simulink library "thc"  (R2021b)
settings: Solver=VariableStepAuto  StartTime=0.0  StopTime=10.0  RelTol=1e-3
undefined symbols (not defined in the file or in its folder): ATHC_APTCQA_X_C, ATHC_APTCQB_X_C, ATHC_dAy_X_C, ATHC_Qeq_X_kmh, ATHC_VbaseC_X_C, ATHC_VbaseC_Y_W, ATHC_VbaseD_X_C, ATHC_VbaseH_X_C, KTHC_ACMaxMinT_sec, KTHC_aDeice_K, KTHC_AGSDefLv_K, KTHC_AGSLv1_K, KTHC_AGSLv2_K, KTHC_AGSLv3_K, KTHC_AGSLv4_K, KTHC_AGSLv5_K, KTHC_AirIntUpdateT_sec, KTHC_APTCOneZoneMax_W, KTHC_APTCPeriod_cnt, KTHC_APTCPWMEN_flg, KTHC_APTCQMaxC_W, KTHC_APTCQminC_W, KTHC_APTCQminD_W, KTHC_APTCQminRe1_W, KTHC_APTCQminRe_W, KTHC_APTCQoffT_cnt, KTHC_APTCQonT_cnt, KTHC_APTCRiLeMaxDff_W, KTHC_APTCRiLeMinDff_W, KTHC_AutoWDTamb1_C, KTHC_AutoWDTamb2_C, KTHC_AutoWDTamb3_C, KTHC_BatCoolT_cnt, KTHC_BatInTempDef_C, KTHC_bDeice_K, KTHC_CompMaxDeice_rpm, KTHC_CompMinDeice_rpm, KTHC_CompSotxvOp_K, KTHC_CompSotxvOpLow_rpm, KTHC_CompSpdEXVUp1_rpm, KTHC_CompSpdEXVUp2_rpm, KTHC_CompSpdEXVUp3_rpm, KTHC_CompSpdEXVUp4_rpm, KTHC_CompSpdmax_rpm, KTHC_CompSpdmaxBC1_rpm, KTHC_CompSpdmaxBC_rpm, KTHC_CompSpdmid1_rpm, KTHC_CompSpdmid2_rpm, KTHC_CompSpdmid3_rpm, KTHC_CompSpdmid4_rpm, KTHC_CompSpdmid5_rpm, KTHC_CompSpdmid_rpm, KTHC_CompSpdmin_rpm, KTHC_DAPTCQ1_W, KTHC_DAPTCQ2_W, KTHC_DAPTCQ3_W, KTHC_DcChSetTemp_C, KTHC_DehumidityEN_flg, KTHC_DeiceCycTime_K, KTHC_DriveLevelWPTCBAH1_W ... (+403)
libraries: simulink x489
(part 3 of 18)

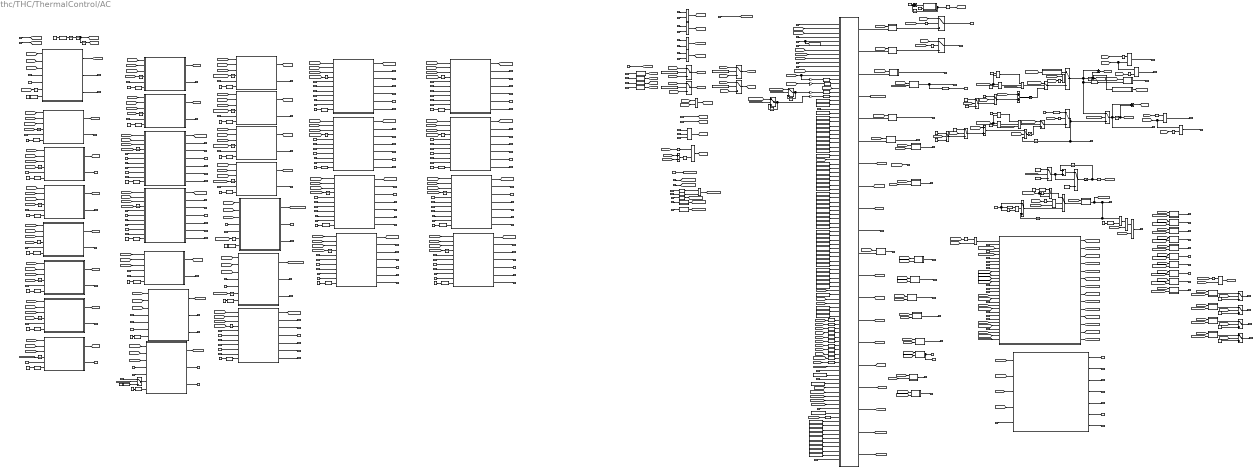
== system thc/THC/ThermalControl/AC ==
  note: PersonalSetting
  VINP_FCPFrEvtBtnACMaxReq_flg : Inport
  VINP_FCPFrEvtBtnACReq_flg : Inport  Port=2
  VINP_FCPFrEvtBtnAutoReq_flg : Inport  Port=3
  VINP_FCPFrEvtBtnSyncReq_flg : Inport  Port=4
  VINP_Tamb_C : Inport  Port=5
  VINP_Tincar_C : Inport  Port=6
  VINP_sigAirIntenZon1Req_enum : Inport  Port=7
  VINP_sigRecircReq_flg : Inport  Port=8
  VINP_sigFaceReq_flg : Inport  Port=9
  VINP_sigFootReq_flg : Inport  Port=10
  VINP_sigFrostReq_flg : Inport  Port=11
  VINP_sigSetTempZon1Req_C : Inport  Port=12
  VINP_CANMsgValidIVI2_flg : Inport  Port=13
  VINP_sigSetTempZon2Req_C : Inport  Port=14
  VTHC_FDBlowerCmd_pct : Inport  Port=15
  PwrSta : Inport  Port=16
  OFF_AC_MODE : Inport  Port=17
  CabinMode : Inport  Port=18
  T_Foot_L : Inport  Port=19
  T_Foot_R : Inport  Port=20
  T_Foot_Rr : Inport  Port=21
  VINP_RemoteAutoReq_flg : Inport  Port=22
  ACSubMode : Inport  Port=23
  EEP_sigSetTempZon2StM : Inport  Port=24
  VINP_HMIACBtnCmd_flg : Inport  Port=25
  VINP_HMIACAutoBtnCmd_flg : Inport  Port=26
  VINP_HMIACRecycleBtnCmd_flg : Inport  Port=27
  VINP_HMIACFrDefogBtnCmd_flg : Inport  Port=28
  VINP_HMIZLSetTPCmd_flg : Inport  Port=29
  VINP_HMIZLSetTMCmd_flg : Inport  Port=30
  VINP_HMIZRSetTPCmd_flg : Inport  Port=31
  VINP_HMIZRSetTMCmd_flg : Inport  Port=32
  VINP_HMIACWindDirPCmd_flg : Inport  Port=33
  VINP_HMIACWindDirMCmd_flg : Inport  Port=34
  VINP_HMIACAirIntPCmd_flg : Inport  Port=35
  VINP_HMIACAirIntMCmd_flg : Inport  Port=36
  VINP_IVIAirIntZ3Cmd_enum : Inport  Port=37
  VINP_IVILBlowerModeSta_enum : Inport  Port=38
  VINP_IVIRBlowerModeSta_enum : Inport  Port=39
  VINP_IVILBlowerZSta_enum : Inport  Port=40
  VINP_IVICLBlowerZSta_enum : Inport  Port=41
  VINP_IVIRBlowerZSta_enum : Inport  Port=42
  VINP_IVICRBlowerZSta_enum : Inport  Port=43
  VINP_IVILBlowerYSta_enum : Inport  Port=44
  VINP_IVICLBlowerYSta_enum : Inport  Port=45
  VINP_IVIRBlowerYSta_enum : Inport  Port=46
  VINP_IVICRBlowerYSta_enum : Inport  Port=47
  VINP_ZFRTHCLEventActYSta_enum : Inport  Port=48
  VINP_ZFRTHCCLEVentActYSta_enum : Inport  Port=49
  VINP_ZFRTHCREventActYSta_enum : Inport  Port=50
  VINP_ZFRTHCCREVentActYSta_enum : Inport  Port=51
  VINP_IVIsigScreenReq_Sta : Inport  Port=52
  VINP_IVIFGSAirIntCmd_enum : Inport  Port=53
  VINP_IVIFGSChCmd_enum : Inport  Port=54
  VINP_IVIIONSWCmd_flg : Inport  Port=55
  VINP_FGSAirIntSta_enum : Inport  Port=56
  VINP_IVIZon1WindDirSWReqSta_flg : Inport  Port=57
  VBCM_UserNow_enum : Inport  Port=58
  VINP_UpdateReq_enum : Inport  Port=59
  EEP_ACModeSet123 : Inport  Port=60
  EEP_ACModeSet457 : Inport  Port=61
  EEP_FACESet : Inport  Port=62
  EEP_FOOTSet : Inport  Port=63
  EEP_FrostSet : Inport  Port=64
  EEP_FaceMSet : Inport  Port=65
  EEP_FootMSet : Inport  Port=66
  EEP_fdefogSet : Inport  Port=67
  EEP_CCUSyncStsSet : Inport  Port=68
  EEP_sigRecircStSet : Inport  Port=69
  EEP_RecyAutoSet : Inport  Port=70
  EEP_AirIntenZone1MSet1 : Inport  Port=71
  EEP_AirIntenZone1MSet2 : Inport  Port=72
  EEP_AirIntenZone1MSet3 : Inport  Port=73
  EEP_AirIntenZone1MSet4 : Inport  Port=74
  EEP_AirIntenZone1MSet5 : Inport  Port=75
  EEP_AirIntenZone1MSet7 : Inport  Port=76
  EEP_AirIntenZone3MSet1 : Inport  Port=77
  EEP_AirIntenZone3MSet2 : Inport  Port=78
  EEP_AirIntenZone3MSet3 : Inport  Port=79
  EEP_AirIntenZone3MSet4 : Inport  Port=80
  EEP_AirIntenZone3MSet5 : Inport  Port=81
  EEP_AirIntenZone3MSet7 : Inport  Port=82
  EEP_IONSWStaSet : Inport  Port=83
  EEP_FDCFGSChStaSet123 : Inport  Port=84
  EEP_FDCFGSChStaSet457 : Inport  Port=85
  EEP_FDCFGSAirIntStaSet123 : Inport  Port=86
  EEP_FDCFGSAirIntStaSet457 : Inport  Port=87
  EEP_LVentENSet : Inport  Port=88
  EEP_CLVentENSet : Inport  Port=89
  EEP_RVentENSet : Inport  Port=90
  EEP_CRVentENSet : Inport  Port=91
  EEP_FDCTHCLEventModeStaSet123 : Inport  Port=92
  EEP_FDCTHCLEventModeStaSet457 : Inport  Port=93
  EEP_FDCTHCREventModeStaSet123 : Inport  Port=94
  EEP_FDCTHCREventModeStaSet457 : Inport  Port=95
  EEP_FDCTHCLEventZStaSet1 : Inport  Port=96
  EEP_FDCTHCLEventZStaSet2 : Inport  Port=97
  EEP_FDCTHCLEventZStaSet3 : Inport  Port=98
  EEP_FDCTHCLEventZStaSet4 : Inport  Port=99
  EEP_FDCTHCLEventZStaSet5 : Inport  Port=100
  EEP_FDCTHCLEventZStaSet7 : Inport  Port=101
  EEP_FDCTHCCLEVentZStaSet1 : Inport  Port=102
  EEP_FDCTHCCLEVentZStaSet2 : Inport  Port=103
  EEP_FDCTHCCLEVentZStaSet3 : Inport  Port=104
  EEP_FDCTHCCLEVentZStaSet4 : Inport  Port=105
  EEP_FDCTHCCLEVentZStaSet5 : Inport  Port=106
  EEP_FDCTHCCLEVentZStaSet7 : Inport  Port=107
  EEP_FDCTHCREventZStaSet1 : Inport  Port=108
  EEP_FDCTHCREventZStaSet2 : Inport  Port=109
  EEP_FDCTHCREventZStaSet3 : Inport  Port=110
  EEP_FDCTHCREventZStaSet4 : Inport  Port=111
  EEP_FDCTHCREventZStaSet5 : Inport  Port=112
  EEP_FDCTHCREventZStaSet7 : Inport  Port=113
  EEP_FDCTHCCREVentZStaSet1 : Inport  Port=114
  EEP_FDCTHCCREVentZStaSet2 : Inport  Port=115
  EEP_FDCTHCCREVentZStaSet3 : Inport  Port=116
  EEP_FDCTHCCREVentZStaSet4 : Inport  Port=117
  EEP_FDCTHCCREVentZStaSet5 : Inport  Port=118
  EEP_FDCTHCCREVentZStaSet7 : Inport  Port=119
  EEP_FDCTHCLEventYStaSet1 : Inport  Port=120
  EEP_FDCTHCLEventYStaSet2 : Inport  Port=121
  EEP_FDCTHCLEventYStaSet3 : Inport  Port=122
  EEP_FDCTHCLEventYStaSet4 : Inport  Port=123
  EEP_FDCTHCLEventYStaSet5 : Inport  Port=124
  EEP_FDCTHCLEventYStaSet7 : Inport  Port=125
  EEP_FDCTHCCLEVentYStaSet1 : Inport  Port=126
  EEP_FDCTHCCLEVentYStaSet2 : Inport  Port=127
  EEP_FDCTHCCLEVentYStaSet3 : Inport  Port=128
  EEP_FDCTHCCLEVentYStaSet4 : Inport  Port=129
  EEP_FDCTHCCLEVentYStaSet5 : Inport  Port=130
  EEP_FDCTHCCLEVentYStaSet7 : Inport  Port=131
  EEP_FDCTHCREventYStaSet1 : Inport  Port=132
  EEP_FDCTHCREventYStaSet2 : Inport  Port=133
  EEP_FDCTHCREventYStaSet3 : Inport  Port=134
  EEP_FDCTHCREventYStaSet4 : Inport  Port=135
  EEP_FDCTHCREventYStaSet5 : Inport  Port=136
  EEP_FDCTHCREventYStaSet7 : Inport  Port=137
  EEP_FDCTHCCREVentYStaSet1 : Inport  Port=138
  EEP_FDCTHCCREVentYStaSet2 : Inport  Port=139
  EEP_FDCTHCCREVentYStaSet3 : Inport  Port=140
  EEP_FDCTHCCREVentYStaSet4 : Inport  Port=141
  EEP_FDCTHCCREVentYStaSet5 : Inport  Port=142
  EEP_FDCTHCCREVentYStaSet7 : Inport  Port=143
  EEP_SettempZon1Set1 : Inport  Port=144
  EEP_SettempZon1Set2 : Inport  Port=145
  EEP_SettempZon1Set3 : Inport  Port=146
  EEP_SettempZon1Set4 : Inport  Port=147
  EEP_SettempZon1Set5 : Inport  Port=148
  EEP_SettempZon1Set7 : Inport  Port=149
  VINP_IVIQuickRefreshSta_flg : Inport  Port=150
  Add{,1..2,5} (4 alike) : Sum
  Add3 : Sum  Inputs=+-
  Add7 : Sum  Inputs=+-
  Add8 : Sum  Inputs=+-
  Chart : Stateflow chart  TreatAsAtomicUnit=on
      settings: PortSchema="{\"entries\":[{\"content\":{\"sides\":[{\"content\":{\"connectorIds\":[\"In1\",\"In2\",\"In3\",\"In4\",\"In5\",\"In6\",\"In7\",\"In8\",\"In9\",\"In10\",\"In11\",\"In12\",\"In13\",\"In14\",\"In15\",\"In16\",\"In18\",\"In17\",\"In19\",\"In20\",\"In21\",\"In22\",\"In23\",\"In24\",\"In25\",\"In26\",\"In27\",\"In28\",\"In29\",\"In30\",\"In31\",\"In32\",\"In33\",\"In34\",\"In35\",\"In36\",\"In37\",\"In38\",\"In39\",\"In40\",\"In41\",\"In42\",\"In43\",\"In44\",\"In45\",\"In46\",\"In47\",\"In48\",\"In49\",\"In50\",\"In51\",\"In52\",\"In53\",\"In54\",\"In55\",\"In56\",\"In57\",\"In58\",\"In59\",\"In60\",\"In61\",\"In62\",\"In63\",\"In64\",\"In65\",\"In66\",\"In67\",\"In68\",\"In69\",\"In70\",\"In71\",\"In72\",\"In73\",\"In74\",\"In75\",\"In76\",\"In77\",\"In78\",\"In79\",\"In80\",\"In81\",\"In82\",\"In83\",\"In84\",\"In85\",\"In86\",\"In87\",\"In88\",\"In89\",\"In90\",\"In91\",\"In92\",\"In93\",\"In94\",\"In95\",\"In96\",\"In97\",\"In98\",\"In99\",\"In100\",\"In101\",\"In102\",\"In103\",\"In104\"]},\"type\":\"ConnectorPlacement.EquallySpacedRectSide\",\"uuid\":\"5820fc40-35f0-4b43-a348-a95be02a5108\"},{\"content\":{\"connectorIds\":[\"Out1\",\"Out6\",\"Out2\",\"Out3\",\"Out4\",\"Out5\",\"Out7\",\"Out8\",\"Out9\",\"Out10\",\"Out11\",\"Out12\",\"Out13\",\"Out14\",\"Out15\",\"Out16\",\"Out17\",\"Out18\",\"Out19\",\"Out20\"],\"side\":\"RIGHT\"},\"type\":\"ConnectorPlacement.EquallySpacedRectSide\",\"uuid\":\"36d6613c-bf09-4a00-b7cd-6c94d14300cf\"},{\"content\":{\"connectorIds\":[],\"side\":\"TOP\"},\"type\":\"ConnectorPlacement.EquallySpacedRectSide\",\"uuid\":\"1ae2c247-46e8-45cc-9ea1-ac445f4d9fda\"}]},\"type\":\"ConnectorPlacement.EquallySpacedConnector\",\"uuid\":\"a8684177-dc23-416a-a392-32f98192c4b4\"}],\"packageUris\":[\"http://schema.mathworks.com/mf0/Connector/R2020b\"],\"version\":\"1.0\"}"
  Compare To Constant : simulink/Logic and Bit Operations/Compare To Constant  relop=<  const=5  OutDataTypeStr=boolean
  Compare To Constant1 : simulink/Logic and Bit Operations/Compare To Constant  relop=>=  const=1  OutDataTypeStr=boolean
  Compare To Constant10 : simulink/Logic and Bit Operations/Compare To Constant  relop=>  const=0  OutDataTypeStr=boolean
  Compare To Constant11 : simulink/Logic and Bit Operations/Compare To Constant  relop=<  const=0  OutDataTypeStr=boolean
  Compare To Constant12 : simulink/Logic and Bit Operations/Compare To Constant  relop=>  const=0  OutDataTypeStr=boolean
  Compare To Constant13 : simulink/Logic and Bit Operations/Compare To Constant  relop=<  const=0  OutDataTypeStr=boolean
  Compare To Constant2 : simulink/Logic and Bit Operations/Compare To Constant  relop=>=  const=100  OutDataTypeStr=boolean
  Compare To Constant3 : simulink/Logic and Bit Operations/Compare To Constant  relop===  const=3.0  OutDataTypeStr=boolean
  Compare To Constant4 : simulink/Logic and Bit Operations/Compare To Constant  relop=<  const=0  OutDataTypeStr=boolean
  Compare To Constant6 : simulink/Logic and Bit Operations/Compare To Constant  relop===  const=2  OutDataTypeStr=boolean
  Compare To Constant7 : simulink/Logic and Bit Operations/Compare To Constant  relop===  const=1  OutDataTypeStr=boolean
  Compare To Constant8 : simulink/Logic and Bit Operations/Compare To Constant  relop===  const=0  OutDataTypeStr=boolean
  Compare To Constant9 : simulink/Logic and Bit Operations/Compare To Constant  relop=>  const=0  OutDataTypeStr=boolean
  Constant{,55,71,80,82,85,91,94,96..101} (14 alike) : Constant
  Constant1 : Constant  Value=10
  Constant10 : Constant  Value=KTHC_T2Mmaxamb_C
  Constant{102..109} (8 alike) : Constant  Value=50
  Constant11 : Constant  Value=KTHC_T3Mmaxamb_C
  Constant{68..70,110} (4 alike) : Constant  Value=KTHC_DriverSeatPos_flg
  Constant111 : Constant  Value=KTHC_AutoWDTamb1_C
  Constant112 : Constant  Value=KTHC_AutoWDTamb2_C
  Constant113 : Constant  Value=KTHC_AutoWDTamb3_C
  Constant114 : Constant  Value=KTHC_WDZ11Foot_flg
  Constant115 : Constant  Value=KTHC_WDZ11Frost_flg
  Constant116 : Constant  Value=KTHC_WDZ11Face_flg
  Constant117 : Constant  Value=KTHC_WDZ12Foot_flg
  Constant118 : Constant  Value=KTHC_WDZ12Frost_flg
  Constant119 : Constant  Value=KTHC_WDZ12Face_flg
  Constant12 : Constant  Value=KTHC_T4Mmaxamb_C
  Constant13 : Constant  Value=KTHC_T3Mminamb_C
  Constant14 : Constant  Value=KTHC_T4Mminamb_C
  Constant15 : Constant  Value=KTHC_T5Mminamb_C
  Constant16 : Constant  Value=KTHC_RecyHold_min
  Constant17 : Constant  Value=KTHC_RecyChange_min
  Constant18 : Constant  Value=KTHC_Tmidlevel_C
  Constant19 : Constant  Value=KTHC_Thilevel1_C
  Constant20 : Constant  Value=KTHC_Thilevel2_C
  Constant21 : Constant  Value=KTHC_WDZ1Face_flg
  Constant22 : Constant  Value=KTHC_WDZ1Foot_flg
  Constant23 : Constant  Value=KTHC_WDZ1Frost_flg
  Constant24 : Constant  Value=KTHC_WDZ2Face_flg
  Constant25 : Constant  Value=KTHC_WDZ2Foot_flg
  Constant26 : Constant  Value=KTHC_WDZ2Frost_flg
  Constant27 : Constant  Value=KTHC_WDZ3Face_flg
  Constant28 : Constant  Value=KTHC_WDZ3Foot_flg
  Constant29 : Constant  Value=KTHC_WDZ3Frost_flg
  Constant30 : Constant  Value=KTHC_WDZ4Face_flg
  Constant31 : Constant  Value=KTHC_WDZ4Foot_flg
  Constant32 : Constant  Value=KTHC_WDZ4Frost_flg
  Constant33 : Constant  Value=KTHC_WDZ5Face_flg
  Constant34 : Constant  Value=KTHC_WDZ5Foot_flg
  Constant35 : Constant  Value=KTHC_WDZ5Frost_flg
  Constant36 : Constant  Value=KTHC_WDZ6Face_flg
  Constant37 : Constant  Value=KTHC_WDZ6Foot_flg
  Constant38 : Constant  Value=KTHC_WDZ6Frost_flg
  Constant39 : Constant  Value=KTHC_WDZ7Face_flg
  Constant4 : Constant  Value=ZERO_INT
  Constant40 : Constant  Value=KTHC_WDZ7Foot_flg
  Constant41 : Constant  Value=KTHC_WDZ7Frost_flg
  Constant42 : Constant  Value=KTHC_WDZ8Face_flg
  Constant43 : Constant  Value=KTHC_WDZ8Foot_flg
  Constant44 : Constant  Value=KTHC_WDZ8Frost_flg
  Constant45 : Constant  Value=KTHC_WDZ9Face_flg
  Constant46 : Constant  Value=KTHC_WDZ9Foot_flg
  Constant47 : Constant  Value=KTHC_WDZ9Frost_flg
  Constant48 : Constant  Value=ONE_INT
  Constant49 : Constant  Value=ZERO_INT
  Constant5 : Constant  Value=KTHC_RecyOutterD_enum
  Constant50 : Constant  Value=KTHC_Trecymin_C
  Constant51 : Constant  Value=KTHC_RefreshEN_flg
  Constant52 : Constant  Value=KTHC_FootColdT_C
  Constant53 : Constant  Value=KTHC_FootColdTdelta_C
  Constant54 : Constant  Value=KTHC_ACMaxMinT_sec
  Constant57 : Constant  Value=KTHC_WDZ10Foot_flg
  Constant58 : Constant  Value=KTHC_WDZ10Frost_flg
  Constant59 : Constant  Value=0.5
  Constant6 : Constant  Value=KTHC_WDZ10Face_flg
  Constant60 : Constant  Value=-0.5
  Constant{61,64,81,83..84,86..90,93,95} (12 alike) : Constant  Value=0
  Constant62 : Constant  Value=0.5
  Constant63 : Constant  Value=-0.5
  Constant65 : Constant  Value=32
  Constant66 : Constant  Value=32
  Constant67 : Constant  Value=7
  Constant7 : Constant  Value=KTHC_WindDirUpdateT_min
  Constant{72..75} (4 alike) : Constant  Value=false
  Constant76 : Constant  Value=4
  Constant77 : Constant  Value=17
  Constant78 : Constant  Value=17
  Constant79 : Constant  Value=KTHC_ScreenUniq_flg
  Constant9 : Constant  Value=KTHC_AirIntUpdateT_sec
  Constant92 : Constant  Value=4
  Data Type Conversion : DataTypeConversion
  Data Type Conversion1 : DataTypeConversion  OutDataTypeStr=single
  Data Type Conversion{6..7,10..11,24..25,27..28,33..43,50} (20 alike) : DataTypeConversion  OutDataTypeStr=uint8
  Data Type Conversion12 : DataTypeConversion  OutDataTypeStr=single
  Data Type Conversion{8..9,13,15..23,26,29..32,44..49,51} (24 alike) : DataTypeConversion  OutDataTypeStr=boolean
  Data Type Conversion{2..5,14} (5 alike) : DataTypeConversion  OutDataTypeStr=uint16
  Detect Change : simulink/Logic and Bit Operations/Detect Change  vinit=0  OutDataTypeStr=boolean
  Detect Change1 : simulink/Logic and Bit Operations/Detect Change  vinit=0  OutDataTypeStr=boolean
  Detect Increase4 : simulink/Logic and Bit Operations/Detect Increase  vinit=0.0  OutDataTypeStr=boolean
  Detect Increase5 : simulink/Logic and Bit Operations/Detect Increase  vinit=0.0  OutDataTypeStr=boolean
  Detect Increase7 : simulink/Logic and Bit Operations/Detect Increase  vinit=0.0  OutDataTypeStr=boolean
  EVent : Subsystem
  Gain{,1..3} (4 alike) : Gain  Gain=10
  HMISwitchReceive : Subsystem
  HMISwitchReceive1 : Subsystem
  HMISwitchReceive2 : Subsystem
  HMISwitchReceive3 : Subsystem
  HMISwitchReceive4 : Subsystem
  HMISwitchReceive5 : Subsystem
  Logical Operator : Logic  Operator=NXOR  AllPortsSameDT=off  OutDataTypeStr=boolean
  Logical Operator{1..2,4..6,11,20..21,23} (9 alike) : Logic  Operator=OR  AllPortsSameDT=off  OutDataTypeStr=boolean
  Logical Operator{3,10,12..16,22} (8 alike) : Logic  AllPortsSameDT=off  OutDataTypeStr=boolean
  Logical Operator{9,25..27} (4 alike) : Logic  Operator=NOT  AllPortsSameDT=off  OutDataTypeStr=boolean
  Logical Operator7 : Logic  Inputs=3  AllPortsSameDT=off  OutDataTypeStr=boolean
  Logical Operator8 : Logic  Inputs=3  AllPortsSameDT=off  OutDataTypeStr=boolean
  Min : MinMax  Inputs=3
  ModMath2 : Subsystem  mask(Count){}
      mask help: Counter function.
      mask Display:
      | fprintf('ModMath');
      | port_label('output', 1, 'Remainder');
      | port_label('input', 1, 'Dividend');
      | port_label('input', 2, 'Divisor');
  RawdataToSettemp : Subsystem
  Relational Operator{,1,4..5} (4 alike) : RelationalOperator  Operator=<=  OutDataTypeStr=boolean  RndMeth=Simplest
  Relational Operator3 : RelationalOperator  Operator=>  OutDataTypeStr=boolean  RndMeth=Simplest
  Saturation : Saturate  UpperLimit=100  LowerLimit=0
  Saturation2 : Saturate  UpperLimit=32  LowerLimit=17
  Saturation3 : Saturate  UpperLimit=32  LowerLimit=17
  SettempToRawData : Subsystem
  Subsystem : Subsystem
  Subsystem1 : Subsystem
  Subsystem10 : Subsystem
  Subsystem11 : Subsystem
  Subsystem12 : Subsystem
  Subsystem13 : Subsystem
  Subsystem14 : Subsystem
  Subsystem15 : Subsystem
  Subsystem16 : Subsystem
  Subsystem17 : Subsystem
  Subsystem18 : Subsystem
  Subsystem19 : Subsystem
  Subsystem2 : Subsystem
  Subsystem20 : Subsystem
  Subsystem21 : Subsystem
  Subsystem22 : Subsystem
  Subsystem23 : Subsystem
  Subsystem24 : Subsystem
  Subsystem25 : Subsystem
  Subsystem26 : Subsystem
  Subsystem27 : Subsystem
  Subsystem28 : Subsystem
  Subsystem29 : Subsystem
  Subsystem3 : Subsystem
  Subsystem30 : Subsystem
  Subsystem31 : Subsystem
  Subsystem32 : Subsystem
  Subsystem33 : Subsystem
  Subsystem4 : Subsystem
  Subsystem5 : Subsystem
  Subsystem6 : Subsystem
  Subsystem7 : Subsystem
  Subsystem8 : Subsystem
  Subsystem9 : Subsystem
  Switch{,1..3,9..32} (28 alike) : Switch  Criteria=u2 > Threshold
  TOGGLE_TYPE_CCUSyncSts : Subsystem
  TOGGLE_TYPE_CLVentEN : Subsystem
  TOGGLE_TYPE_CRVentEN : Subsystem
  TOGGLE_TYPE_FACE : Subsystem
  TOGGLE_TYPE_FACEM : Subsystem
  TOGGLE_TYPE_FOOT : Subsystem
  TOGGLE_TYPE_FOOTM : Subsystem
  TOGGLE_TYPE_FROST : Subsystem
  TOGGLE_TYPE_IONSWSta : Subsystem
  TOGGLE_TYPE_LVentEN : Subsystem
  TOGGLE_TYPE_RVentEN : Subsystem
  TOGGLE_TYPE_RecyAutoFlg : Subsystem
  TOGGLE_TYPE_fdefog : Subsystem
  TOGGLE_TYPE_sigRecircSt : Subsystem
  Unit Delay1 : UnitDelay  InitialCondition=26  SampleTime=-1  HasFrameUpgradeWarning=on
  Unit Delay{2..38} (37 alike) : UnitDelay  SampleTime=-1  HasFrameUpgradeWarning=on
  VALUE_TYPE_ACModeMem : Subsystem
  VALUE_TYPE_AirIntenZone1M : Subsystem
  VALUE_TYPE_AirIntenZone3M : Subsystem
  VALUE_TYPE_FDCFGSAirIntSta : Subsystem
  VALUE_TYPE_FDCFGSChStaSet : Subsystem
  VALUE_TYPE_FDCTHCCLEVentYSta : Subsystem
  VALUE_TYPE_FDCTHCCLEVentZSta : Subsystem
  VALUE_TYPE_FDCTHCCREVentYSta : Subsystem
  VALUE_TYPE_FDCTHCCREVentZSta : Subsystem
  VALUE_TYPE_FDCTHCLEventYSta : Subsystem
  VALUE_TYPE_FDCTHCLEventZSta : Subsystem
  VALUE_TYPE_FDCTHCREventYSta : Subsystem
  VALUE_TYPE_FDCTHCREventZSta : Subsystem
  VALUE_TYPE_LEventModeSta : Subsystem
  VALUE_TYPE_REventModeSta : Subsystem
  VALUE_TYPE_SettempZon1 : Subsystem
  VTHC_CCUACLampSts_flg : Outport
  VTHC_CCUAutoLampSts_flg : Outport  Port=2
  VTHC_CCUACMaxLampSts_flg : Outport  Port=3
  VTHC_CCUSyncLampSts_flg : Outport  Port=4
  VTHC_sigAirIntenZon1St_enum : Outport  Port=5
  VTHC_sigWindDirZon1St_enum : Outport  Port=6
  VTHC_sigRecircSt_flg : Outport  Port=7
  VTHC_sigSetTempZon1St_C : Outport  Port=8
  VTHC_sigSetTempZon2St_C : Outport  Port=9
  WaterFillReq : Outport  Port=10
  PET : Outport  Port=11
  FD_RecyAuto_Cmd : Outport  Port=12
  ACModeMem : Outport  Port=13
  Face : Outport  Port=14
  Foot : Outport  Port=15
  Frost : Outport  Port=16
  FaceM : Outport  Port=17
  FootM : Outport  Port=18
  CCUSyncSts : Outport  Port=19
  RecAutoFlg : Outport  Port=20
  AirIntenZone1M : Outport  Port=21
  fdefog : Outport  Port=22
  VTHC_sigSetTempZon2StM_C : Outport  Port=23
  VTHC_sigDfrstSt_flg : Outport  Port=24
  VTHC_FDCTHCAirIntZ3Sta_enum : Outport  Port=25
  RrAPTCEN : Outport  Port=26
  VTHC_FDCTHCLEventModeSta_enum : Outport  Port=27
  VTHC_FDCTHCREventModeSta_enum : Outport  Port=28
  VTHC_FDCTHCLEventZSta_enum : Outport  Port=29
  VTHC_FDCTHCCLEVentZSta_enum : Outport  Port=30
  VTHC_FDCTHCREventZSta_enum : Outport  Port=31
  VTHC_FDCTHCCREVentZSta_enum : Outport  Port=32
  VTHC_FDCTHCLEventYSta_enum : Outport  Port=33
  VTHC_FDCTHCLVentENSta_flg : Outport  Port=34
  VTHC_FDCTHCCLEVentYSta_enum : Outport  Port=35
  VTHC_FDCTHCCLVentENSta_flg : Outport  Port=36
  VTHC_FDCTHCREventYSta_enum : Outport  Port=37
  VTHC_FDCTHCRVentENSta_flg : Outport  Port=38
  VTHC_FDCTHCCREVentYSta_enum : Outport  Port=39
  VTHC_FDCTHCCRVentENSta_flg : Outport  Port=40
  VTHC_Z1TUP_flg : Outport  Port=41
  VTHC_Z1TDN_flg : Outport  Port=42
  VTHC_Z2TUP_flg : Outport  Port=43
  VTHC_Z2TDN_flg : Outport  Port=44
  VTHC_FDCFGSAirIntSta_enum : Outport  Port=45
  VTHC_FDCFGSChSta_enum : Outport  Port=46
  VTHC_FDCFGSAirIntCmd_enum : Outport  Port=47
  VTHC_FDCFGSFuncSta_enum : Outport  Port=48
  VTHC_FDCFGSChCmd_enum : Outport  Port=49
  VTHC_FDCFGSIONSWSta_flg : Outport  Port=50
  VTHC_FDCFGSIONCmd_flg : Outport  Port=51
  ACModeSet123 : Outport  Port=52
  ACModeSet457 : Outport  Port=53
  FACESet : Outport  Port=54
  FOOTSet : Outport  Port=55
  FrostSet : Outport  Port=56
  FaceMSet : Outport  Port=57
  FootMSet : Outport  Port=58
  fdefogSet : Outport  Port=59
  CCUSyncStsSet : Outport  Port=60
  sigRecircStSet : Outport  Port=61
  RecyAutoSet : Outport  Port=62
  AirIntenZone1MSet1 : Outport  Port=63
  AirIntenZone1MSet2 : Outport  Port=64
  AirIntenZone1MSet3 : Outport  Port=65
  AirIntenZone1MSet4 : Outport  Port=66
  AirIntenZone1MSet5 : Outport  Port=67
  AirIntenZone1MSet7 : Outport  Port=68
  AirIntenZone3MSet1 : Outport  Port=69
  AirIntenZone3MSet2 : Outport  Port=70
  AirIntenZone3MSet3 : Outport  Port=71
  AirIntenZone3MSet4 : Outport  Port=72
  AirIntenZone3MSet5 : Outport  Port=73
  AirIntenZone3MSet7 : Outport  Port=74
  IONSWStaSet : Outport  Port=75
  FDCFGSChStaSet123 : Outport  Port=76
  FDCFGSChStaSet457 : Outport  Port=77
  FDCFGSAirIntStaSet123 : Outport  Port=78
  FDCFGSAirIntStaSet457 : Outport  Port=79
  LVentENSet : Outport  Port=80
  CLVentENSet : Outport  Port=81
  RVentENSet : Outport  Port=82
  CRVentENSet : Outport  Port=83
  FDCTHCLEventModeStaSet123 : Outport  Port=84
  FDCTHCLEventModeStaSet457 : Outport  Port=85
  FDCTHCREventModeStaSet123 : Outport  Port=86
  FDCTHCREventModeStaSet457 : Outport  Port=87
  FDCTHCLEventZStaSet1 : Outport  Port=88
  FDCTHCLEventZStaSet2 : Outport  Port=89
  FDCTHCLEventZStaSet3 : Outport  Port=90
  FDCTHCLEventZStaSet4 : Outport  Port=91
  FDCTHCLEventZStaSet5 : Outport  Port=92
  FDCTHCLEventZStaSet7 : Outport  Port=93
  FDCTHCCLEVentZStaSet1 : Outport  Port=94
  FDCTHCCLEVentZStaSet2 : Outport  Port=95
  FDCTHCCLEVentZStaSet3 : Outport  Port=96
  FDCTHCCLEVentZStaSet4 : Outport  Port=97
  FDCTHCCLEVentZStaSet5 : Outport  Port=98
  FDCTHCCLEVentZStaSet7 : Outport  Port=99
  FDCTHCREventZStaSet1 : Outport  Port=100
  FDCTHCREventZStaSet2 : Outport  Port=101
  FDCTHCREventZStaSet3 : Outport  Port=102
  FDCTHCREventZStaSet4 : Outport  Port=103
  FDCTHCREventZStaSet5 : Outport  Port=104
  FDCTHCREventZStaSet7 : Outport  Port=105
  FDCTHCCREVentZStaSet1 : Outport  Port=106
  FDCTHCCREVentZStaSet2 : Outport  Port=107
  FDCTHCCREVentZStaSet3 : Outport  Port=108
  FDCTHCCREVentZStaSet4 : Outport  Port=109
  FDCTHCCREVentZStaSet5 : Outport  Port=110
  FDCTHCCREVentZStaSet7 : Outport  Port=111
  FDCTHCLEventYStaSet1 : Outport  Port=112
  FDCTHCLEventYStaSet2 : Outport  Port=113
  FDCTHCLEventYStaSet3 : Outport  Port=114
  FDCTHCLEventYStaSet4 : Outport  Port=115
  FDCTHCLEventYStaSet5 : Outport  Port=116
  FDCTHCLEventYStaSet7 : Outport  Port=117
  FDCTHCCLEVentYStaSet1 : Outport  Port=118
  FDCTHCCLEVentYStaSet2 : Outport  Port=119
  FDCTHCCLEVentYStaSet3 : Outport  Port=120
  FDCTHCCLEVentYStaSet4 : Outport  Port=121
  FDCTHCCLEVentYStaSet5 : Outport  Port=122
  FDCTHCCLEVentYStaSet7 : Outport  Port=123
  FDCTHCREventYStaSet1 : Outport  Port=124
  FDCTHCREventYStaSet2 : Outport  Port=125
  FDCTHCREventYStaSet3 : Outport  Port=126
  FDCTHCREventYStaSet4 : Outport  Port=127
  FDCTHCREventYStaSet5 : Outport  Port=128
  FDCTHCREventYStaSet7 : Outport  Port=129
  FDCTHCCREVentYStaSet1 : Outport  Port=130
  FDCTHCCREVentYStaSet2 : Outport  Port=131
  FDCTHCCREVentYStaSet3 : Outport  Port=132
  FDCTHCCREVentYStaSet4 : Outport  Port=133
  FDCTHCCREVentYStaSet5 : Outport  Port=134
  FDCTHCCREVentYStaSet7 : Outport  Port=135
  SettempZon1Set1 : Outport  Port=136
  SettempZon1Set2 : Outport  Port=137
  SettempZon1Set3 : Outport  Port=138
  SettempZon1Set4 : Outport  Port=139
  SettempZon1Set5 : Outport  Port=140
  SettempZon1Set7 : Outport  Port=141
  wires:
  Logical Operator16/1 -> VTHC_Z2TDN_flg/1  "VTHC_Z2TDN_flg"
  [Z2TempG] -> Compare To Constant13/1
  Logical Operator15/1 -> VTHC_Z2TUP_flg/1  "VTHC_Z2TUP_flg"
  Compare To Constant13/1 -> Logical Operator16/2
  Compare To Constant12/1 -> Logical Operator15/1
  [Z2TempG] -> Compare To Constant12/1
  Add8/1 -> [Z2TempG]
  [fInitial] -> Logical Operator16/1, Logical Operator15/2
  Logical Operator14/1 -> VTHC_Z1TDN_flg/1  "VTHC_Z1TDN_flg"
  [Z1TempG] -> Compare To Constant11/1
  Unit Delay10/1 -> SettempToRawData/1(TempIN), [sigSetTempZon1St], Add7/2
  Switch11/1 -> Add7/1, Switch/1, Data Type Conversion12/1, Unit Delay10/1  "VTHC_sigSetTempZon1St_C"
  Add7/1 -> [Z1TempG]
  Compare To Constant11/1 -> Logical Operator14/2
  Compare To Constant10/1 -> Logical Operator13/1
  Logical Operator13/1 -> VTHC_Z1TUP_flg/1  "VTHC_Z1TUP_flg"
  [fInitial] -> Logical Operator14/1, Logical Operator13/2
  [Z1TempG] -> Compare To Constant10/1
  Subsystem33/1(DataOut) -> VTHC_sigSetTempZon1St_C/1  "VTHC_sigSetTempZon1St_C"
  VINP_IVIsigScreenReq_Sta/1 -> Chart/92(sigScreenReq)
  Logical Operator12/1 -> [EVACEN]
  [Face] -> Logical Operator12/2
  Compare To Constant9/1 -> Logical Operator12/1
  [VTHC_FDBlowerCmd_pct] -> Compare To Constant9/1
  Constant76/1 -> Data Type Conversion11/1
  Data Type Conversion11/1 -> Switch29/1
  [EEP_AirIntenZone3M] -> Compare To Constant8/1, Switch29/3
  Compare To Constant8/1 -> Switch29/2
  [EVACEN] -> Switch28/2
  Constant75/1 -> Switch28/3
  Constant74/1 -> Switch27/3
  [EVACEN] -> Switch27/2
  [EVACEN] -> Switch26/2
  Constant73/1 -> Switch26/3
  Constant72/1 -> Switch25/3
  [EVACEN] -> Switch25/2
  Switch25/1 -> VTHC_FDCTHCLVentENSta_flg/1
  Switch28/1 -> VTHC_FDCTHCCRVentENSta_flg/1
  Switch27/1 -> VTHC_FDCTHCRVentENSta_flg/1
  Switch26/1 -> VTHC_FDCTHCCLVentENSta_flg/1
  Logical Operator11/1 -> RrAPTCEN/1
  [Foot] -> Logical Operator11/2
  Logical Operator10/1 -> Logical Operator11/1
  Relational Operator3/1 -> Logical Operator10/1
  [Face] -> Logical Operator10/2
  Data Type Conversion10/1 -> Relational Operator3/2
  Constant71/1 -> Data Type Conversion10/1
  [EEP_FDCTHCCREVentYSta] -> EVent/29(VINP_FDCTHCCREVentYStaM_enum)
  [EEP_CRVentEN] -> EVent/28(VTHC_FDCTHCCRVentENM_flg)
  [EEP_FDCTHCREventYSta] -> EVent/26(VINP_FDCTHCREventYStaM_enum)
  [EEP_RVentEN] -> EVent/25(VTHC_FDCTHCRVentENM_flg)
  [EEP_FDCTHCCLEVentYSta] -> EVent/21(VINP_FDCTHCCLEVentYStaM_enum)
  [EEP_CLVentEN] -> EVent/20(VTHC_FDCTHCCLVentENM_flg)
  [EEP_FDCTHCLEventYSta] -> EVent/18(VINP_FDCTHCLEventYStaM_enum)
  [EEP_LVentEN] -> EVent/17(VTHC_FDCTHCLVentENM_flg)
  [EEP_FDCTHCCREVentZSta] -> EVent/13(VINP_FDCTHCCREVentZStaM_enum)
  [EEP_FDCTHCREventZSta] -> EVent/12(VINP_FDCTHCREventZStaM_enum)
  [EEP_FDCTHCCLEVentZSta] -> EVent/11(VINP_FDCTHCCLEVentZStaM_enum)
  [EEP_FDCTHCLEventZSta] -> EVent/10(VINP_FDCTHCLEventZStaM_enum)
  VINP_ZFRTHCCREVentActYSta_enum/1 -> EVent/27(VINP_ZFRTHCCREVentActYSta_enum)
  VINP_ZFRTHCREventActYSta_enum/1 -> EVent/24(VINP_ZFRTHCREventActYSta_enum)
  VINP_ZFRTHCCLEVentActYSta_enum/1 -> EVent/19(VINP_ZFRTHCCLEVentActYSta_enum)
  VINP_ZFRTHCLEventActYSta_enum/1 -> EVent/16(VINP_ZFRTHCLEventActYSta_enum)
  VINP_IVICRBlowerYSta_enum/1 -> EVent/23(VINP_IVICRBlowerYSta_enum)
  VINP_IVIRBlowerYSta_enum/1 -> EVent/22(VINP_IVIRBlowerYSta_enum)
  VINP_IVICLBlowerYSta_enum/1 -> EVent/15(VINP_IVICLBlowerYSta_enum)
  VINP_IVILBlowerYSta_enum/1 -> EVent/14(VINP_IVILBlowerYSta_enum)
  VINP_IVICRBlowerZSta_enum/1 -> EVent/9(VINP_IVICRBlowerZSta_enum)
  VINP_IVIRBlowerZSta_enum/1 -> EVent/8(VINP_IVIRBlowerZSta_enum)
  VINP_IVICLBlowerZSta_enum/1 -> EVent/7(VINP_IVICLBlowerZSta_enum)
  VINP_IVILBlowerZSta_enum/1 -> EVent/6(VINP_IVILBlowerZSta_enum)
  VINP_IVIRBlowerModeSta_enum/1 -> EVent/4(VINP_IVIRBlowerModeSta_enum)
  VINP_IVILBlowerModeSta_enum/1 -> EVent/2(VINP_IVILBlowerModeSta_enum)
  Subsystem18/1(DataOut) -> [AirIntenZone3M], VTHC_FDCTHCAirIntZ3Sta_enum/1, Unit Delay9/1, Relational Operator3/1  "VTHC_FDCTHCAirIntZ3Sta_enum"
  Switch23/1 -> Switch24/3
  Switch29/1 -> Switch24/1
  Unit Delay9/1 -> Switch23/3
  Compare To Constant1/1 -> Logical Operator3/2
  Logical Operator3/1 -> Switch23/2
  Detect Change/1 -> Logical Operator3/1
  VINP_IVIAirIntZ3Cmd_enum/1 -> Detect Change/1, Compare To Constant1/1, Switch23/1
  [sigAirIntenZon1Req] -> Chart/8(sigAirIntenZon1Req)
  VINP_sigAirIntenZon1Req_enum/1 -> [sigAirIntenZon1Req]
  HMISwitchReceive5/1(Out1) -> [AirIntM]
  [AirIntM] -> Chart/91(AirIntM)
  [AirIntP] -> Chart/90(AirIntP)
  [WindDirM] -> Chart/89(WindDirM)
  [WindDirP] -> Chart/88(WindDirP)
  HMISwitchReceive4/1(Out1) -> [AirIntP]
  Detect Increase5/1 -> [WindDirM]
  Detect Increase4/1 -> Logical Operator20/1
  VINP_HMIACAirIntPCmd_flg/1 -> HMISwitchReceive4/1(In1)
  VINP_HMIACAirIntMCmd_flg/1 -> HMISwitchReceive5/1(In1)
  VINP_HMIACWindDirMCmd_flg/1 -> Detect Increase5/1
  VINP_HMIACWindDirPCmd_flg/1 -> Detect Increase4/1
  [VINP_sigSetTempZon2Req_C] -> Relational Operator4/2, Relational Operator1/1
  Constant66/1 -> Relational Operator1/2
  Relational Operator1/1 -> Logical Operator8/2
  [VINP_CANMsgValidIVI2_flg] -> Logical Operator8/3
  Logical Operator8/1 -> Switch2/2
  [VINP_sigSetTempZon2Req_C] -> Switch2/1
  [VINP_sigSetTempZon1Req_C] -> Switch1/1
  Constant65/1 -> Relational Operator/2
  Relational Operator/1 -> Logical Operator7/2
  Logical Operator7/1 -> Switch1/2
  Saturation3/1 -> Switch2/3
  Saturation2/1 -> Switch1/3
  Switch20/1 -> Saturation3/1
  [SyncCancel] -> Switch20/2
  Add5/1 -> Switch20/1
  Unit Delay1/1 -> Switch20/3
  [sigSetTempZon2St] -> Add5/1
  [Z2SetTP] -> Switch18/2
  Constant62/1 -> Switch18/1
  Switch19/1 -> Switch18/3
  Switch18/1 -> Add5/2
  [Z2SetTM] -> Switch19/2
  Constant63/1 -> Switch19/1
  Constant64/1 -> Switch19/3
  Constant61/1 -> Switch17/3
  Constant60/1 -> Switch17/1
  [Z1SetTM] -> Switch17/2
  Switch16/1 -> Add1/2
  Switch17/1 -> Switch16/3
  Constant59/1 -> Switch16/1
  [Z1SetTP] -> Switch16/2
  Add1/1 -> Saturation2/1
  [sigSetTempZon1St] -> Add1/1
  [VINP_CANMsgValidIVI2_flg] -> Switch9/2
  [VINP_CANMsgValidIVI2_flg] -> Logical Operator7/3
  [SyncCancel] -> Chart/87(SyncCancel)
  Logical Operator6/1 -> [SyncCancel]
  [Z2SetTM] -> Logical Operator6/2
  [Z2SetTP] -> Logical Operator6/1
  HMISwitchReceive2/1(Out1) -> [ZRSetTP]
  HMISwitchReceive3/1(Out1) -> [ZRSetTM]
  HMISwitchReceive1/1(Out1) -> [ZLSetTM]
  HMISwitchReceive/1(Out1) -> [ZLSetTP]
  [FrDefogBtn] -> Chart/12(sigFrostReq)
  Logical Operator5/1 -> [FrDefogBtn]
  VINP_sigFrostReq_flg/1 -> Logical Operator5/1
  VINP_HMIACFrDefogBtnCmd_flg/1 -> Logical Operator5/2
  [RecycleBtn] -> Chart/9(sigRecircReq)
  Logical Operator4/1 -> [RecycleBtn]
  VINP_sigRecircReq_flg/1 -> Logical Operator4/1
  VINP_HMIACRecycleBtnCmd_flg/1 -> Logical Operator4/2
  VINP_FCPFrEvtBtnSyncReq_flg/1 -> Chart/4(FCP_FrEvt_BtnSyncReq)
  [ACAUTOBtn] -> Chart/3(FCP_FrEvt_BtnAutoReq)
  Logical Operator2/1 -> [ACAUTOBtn]
  VINP_HMIACAutoBtnCmd_flg/1 -> Logical Operator2/2
  VINP_FCPFrEvtBtnAutoReq_flg/1 -> Logical Operator2/1
  [ACBtn] -> Chart/2(FCP_FrEvt_BtnACReq)
  Logical Operator1/1 -> [ACBtn]
  VINP_HMIACBtnCmd_flg/1 -> Logical Operator1/2
  VINP_FCPFrEvtBtnACReq_flg/1 -> Logical Operator1/1
  Constant58/1 -> Chart/63(KTHC_WDZ10Frost_flg)
  Constant57/1 -> Chart/62(KTHC_WDZ10Foot_flg)
  Constant6/1 -> Chart/61(KTHC_WDZ10Face_flg)
  [VINP_CANMsgValidIVI2_flg] -> Switch15/2
  [VINP_sigSetTempZon2Req_C] -> Switch15/1
  Unit Delay8/1 -> Switch15/3
  Switch15/1 -> Unit Delay8/1, Gain3/1
  [VINP_CANMsgValidIVI2_flg] -> Switch14/2
  Unit Delay5/1 -> Switch14/3
  [VINP_sigSetTempZon1Req_C] -> Switch14/1
  Constant5/1 -> Chart/86(KTHC_RecyOutterD_enum)
  Data Type Conversion5/1 -> Chart/17(sigSetTempZon2Req_CMD)
  Gain3/1 -> Data Type Conversion5/1
  Gain2/1 -> Data Type Conversion4/1
  Data Type Conversion4/1 -> Chart/18(sigSetTempZon1Req_CMD)
  Switch14/1 -> Gain2/1, Unit Delay5/1
  ACSubMode/1 -> Chart/85(ACSubMode)
  Constant50/1 -> Chart/84(KTHC_Trecymin_C)
  Compare To Constant7/1 -> Switch3/2
  Compare To Constant6/1 -> Switch13/2
  [WaterFillReq] -> Compare To Constant6/1
  Switch13/1 -> VTHC_CCUAutoLampSts_flg/1  "VTHC_CCUAutoLampSts_flg"
  [Flash] -> Switch13/1
  [Flash] -> Switch3/1
  Compare To Constant/1 -> [Flash]
  Subsystem4/1(DataOut) -> Switch13/3  "VTHC_CCUAutoLampSts_flg"
  VINP_RemoteAutoReq_flg/1 -> Chart/83(VINP_RemoteAutoReq_flg)
  Gain1/1 -> Data Type Conversion3/1
  [sigSetTempZon2St] -> Gain1/1
  Data Type Conversion3/1 -> Chart/15(SetTempZon2St_CMD)
  [sigSetTempZon1St] -> Gain/1, Chart/13(sigSetTempZon1St)
  Data Type Conversion2/1 -> Chart/14(SetTempZon1St_CMD)
  Gain/1 -> Data Type Conversion2/1
  EEP_sigSetTempZon2StM/1 -> Data Type Conversion1/1
  RawdataToSettemp/1(TempOut) -> Switch11/1
  ModMath2/1(Remainder) -> Compare To Constant/1, Unit Delay4/1
  Unit Delay7/1 -> [sigSetTempZon2St], Add8/2
  [VINP_CANMsgValidIVI2_flg] -> Chart/82(VINP_CANMsgValidIVI2_flg)
  [fInitial] -> Logical Operator25/1
  Switch2/1 -> Switch12/3
  Logical Operator23/1 -> Switch11/2
  Switch1/1 -> Switch11/3
  Chart/19(AirIntenZone1M) -> [AirIntenZone1M]
  Subsystem16/1(DataOut) -> RecAutoFlg/1
  Subsystem15/1(DataOut) -> VTHC_sigDfrstSt_flg/1, fdefog/1  "VTHC_sigDfrstSt_flg"
  [EEP_fdefog] -> Data Type Conversion51/1
  Subsystem14/1(DataOut) -> Foot/1
  Subsystem13/1(DataOut) -> Face/1
  Chart/13(FaceM) -> [FaceM]
  Chart/12(ACModeMem) -> [ACMode]
  [EEP_AirIntenZone1M] -> Data Type Conversion50/1
  [EEP_RecyAutoFlg] -> Data Type Conversion49/1
  [EEP_sigRecircSt] -> Data Type Conversion48/1
  [EEP_CCUSyncSts] -> Data Type Conversion47/1
  [EEP_FootM] -> Data Type Conversion46/1
  [EEP_FaceM] -> Data Type Conversion45/1
  [EEP_Frost] -> Data Type Conversion44/1
  [EEP_FOOT] -> Data Type Conversion9/1
  [EEP_FACE] -> Data Type Conversion8/1
  Constant54/1 -> Chart/70(KTHC_ACMaxMinT_sec)
  [MaxFinish] -> Chart/66(MaxFinish)
  Logical Operator/1 -> [MaxFinish]
  Compare To Constant4/1 -> Logical Operator/2
  Compare To Constant3/1 -> Logical Operator/1
  Add3/1 -> Compare To Constant4/1
  [sigSetTempZon1St] -> Add3/2
  [Tincar] -> Add3/1
  [Tincar] -> Chart/7(Tincar)
  VINP_Tincar_C/1 -> [Tincar]
  [CabinMode] -> Compare To Constant3/1
  [CabinMode] -> Chart/33(CabinMode)
  CabinMode/1 -> [CabinMode]
  Constant53/1 -> Chart/69(KTHC_FootColdTdelta_C)
  Constant52/1 -> Chart/68(KTHC_FootColdT_C)
  [T_Foot_min] -> Chart/67(T_Foot_min)
  Min/1 -> [T_Foot_min]
  T_Foot_Rr/1 -> Min/3
  T_Foot_R/1 -> Min/2
  T_Foot_L/1 -> Min/1
  Constant51/1 -> Chart/65(KTHC_RefreshEN_flg)
  [ForceAuto] -> Chart/64(ForceAuto)
  Compare To Constant2/1 -> [ForceAuto]
  Saturation/1 -> Unit Delay6/1, Compare To Constant2/1
  Unit Delay6/1 -> Add2/1
  Switch10/1 -> Saturation/1
  Constant4/1 -> Switch10/3
  Add2/1 -> Switch10/1
  Switch9/1 -> Add2/2, Switch10/2
  Constant48/1 -> Switch9/3
  Constant49/1 -> Switch9/1
  Constant47/1 -> Chart/60(KTHC_WDZ9Frost_flg)
  Constant46/1 -> Chart/59(KTHC_WDZ9Foot_flg)
  Constant45/1 -> Chart/58(KTHC_WDZ9Face_flg)
  Constant44/1 -> Chart/57(KTHC_WDZ8Frost_flg)
  Constant43/1 -> Chart/56(KTHC_WDZ8Foot_flg)
  Constant42/1 -> Chart/55(KTHC_WDZ8Face_flg)
  Constant41/1 -> Chart/54(KTHC_WDZ7Frost_flg)
  Constant40/1 -> Chart/53(KTHC_WDZ7Foot_flg)
  Constant39/1 -> Chart/52(KTHC_WDZ7Face_flg)
  Constant38/1 -> Chart/51(KTHC_WDZ6Frost_flg)
  Constant37/1 -> Chart/50(KTHC_WDZ6Foot_flg)
  Constant36/1 -> Chart/49(KTHC_WDZ6Face_flg)
  Constant35/1 -> Chart/48(KTHC_WDZ5Frost_flg)
  Constant34/1 -> Chart/47(KTHC_WDZ5Foot_flg)
  Constant33/1 -> Chart/46(KTHC_WDZ5Face_flg)
  Constant32/1 -> Chart/45(KTHC_WDZ4Frost_flg)
  Constant31/1 -> Chart/44(KTHC_WDZ4Foot_flg)
  Constant30/1 -> Chart/43(KTHC_WDZ4Face_flg)
  Constant29/1 -> Chart/42(KTHC_WDZ3Frost_flg)
  Constant28/1 -> Chart/41(KTHC_WDZ3Foot_flg)
  Constant27/1 -> Chart/40(KTHC_WDZ3Face_flg)
  Constant26/1 -> Chart/39(KTHC_WDZ2Frost_flg)
  Constant25/1 -> Chart/38(KTHC_WDZ2Foot_flg)
  Constant24/1 -> Chart/37(KTHC_WDZ2Face_flg)
  Constant22/1 -> Chart/35(KTHC_WDZ1Foot_flg)
  Constant23/1 -> Chart/36(KTHC_WDZ1Frost_flg)
  Constant21/1 -> Chart/34(KTHC_WDZ1Face_flg)
  Constant20/1 -> Chart/32(KTHC_Thilevel2_C)
  Constant19/1 -> Chart/31(KTHC_Thilevel1_C)
  Constant18/1 -> Chart/30(KTHC_Tmidlevel_C)
  Constant17/1 -> Chart/29(KTHC_RecyChange_min)
  Constant16/1 -> Chart/28(KTHC_RecyHold_min)
  Constant15/1 -> Chart/27(KTHC_T5Mminamb_C)
  Constant14/1 -> Chart/26(KTHC_T4Mminamb_C)
  Constant13/1 -> Chart/25(KTHC_T3Mminamb_C)
  Constant12/1 -> Chart/24(KTHC_T4Mmaxamb_C)
  Constant11/1 -> Chart/23(KTHC_T3Mmaxamb_C)
  Constant10/1 -> Chart/22(KTHC_T2Mmaxamb_C)
  Chart/10(PET) -> PET/1
  OFF_AC_MODE/1 -> Chart/21(OFF_AC_MODE)
  Constant9/1 -> Chart/20(KTHC_AirIntUpdateT_sec)
  VINP_sigSetTempZon1Req_C/1 -> [VINP_sigSetTempZon1Req_C]
  VINP_sigSetTempZon2Req_C/1 -> [VINP_sigSetTempZon2Req_C]
  Subsystem1/1(DataOut) -> VTHC_sigAirIntenZon1St_enum/1  "VTHC_sigAirIntenZon1St_enum"
  Constant7/1 -> Chart/19(KTHC_WindDirUpdateT_min)
  Subsystem2/1(DataOut) -> VTHC_CCUSyncLampSts_flg/1, Data Type Conversion/1  "VTHC_CCUSyncLampSts_flg"
  Switch3/1 -> VTHC_CCUACLampSts_flg/1  "VTHC_CCUACLampSts_flg"
  Subsystem3/1(DataOut) -> VTHC_CCUACMaxLampSts_flg/1  "VTHC_CCUACMaxLampSts_flg"
  Subsystem5/1(DataOut) -> Switch3/3
  [WaterFillReq] -> Compare To Constant7/1
  Constant1/1 -> ModMath2/2(Divisor)
  Constant/1 -> Add/1
  Unit Delay4/1 -> Add/2
  Add/1 -> ModMath2/1(Dividend)
  Chart/8(WaterFillReq) -> [WaterFillReq]
  [Frost] -> Subsystem8/2(DataIn)
  VTHC_FDBlowerCmd_pct/1 -> Chart/5(FD_Blower_Cmd), [VTHC_FDBlowerCmd_pct]
  VINP_CANMsgValidIVI2_flg/1 -> [VINP_CANMsgValidIVI2_flg]  "VINP_CANMsgValidIVI2_flg"
  VINP_sigFootReq_flg/1 -> Chart/11(sigFootReq)
  VINP_sigFaceReq_flg/1 -> Chart/10(sigFaceReq)
  Subsystem6/1(DataOut) -> VTHC_sigWindDirZon1St_enum/1  "VTHC_sigWindDirZon1St_enum"
  VINP_FCPFrEvtBtnACMaxReq_flg/1 -> Chart/1(FCP_FrEvt_BtnACMaxReq)
  Subsystem7/1(DataOut) -> VTHC_sigRecircSt_flg/1  "VTHC_sigRecircSt_flg"
  VINP_Tamb_C/1 -> Chart/6(Tamb)
  [VTHC_CCUSyncSts_flg] -> Switch/2
  Constant77/1 -> Relational Operator4/1
  Relational Operator4/1 -> Logical Operator8/1
  Relational Operator5/1 -> Logical Operator7/1
  Constant78/1 -> Relational Operator5/1
  [VINP_sigSetTempZon1Req_C] -> Relational Operator5/2, Relational Operator/1
  PwrSta/1 -> [PwrSta]
  [PwrSta] -> Chart/16(PwrSta)
  [PwrSta] -> Subsystem/3(PwrSta)
  VINP_FGSAirIntSta_enum/1 -> Subsystem/5(FGS_AirInt_Sta)
  Subsystem/1(FGSAirIntSta) -> VTHC_FDCFGSAirIntSta_enum/1
  Subsystem/2(FGSChSta) -> VTHC_FDCFGSChSta_enum/1
  Subsystem/3(FGSAirIntCmd) -> VTHC_FDCFGSAirIntCmd_enum/1
  Subsystem/4(FGSFuncSta) -> VTHC_FDCFGSFuncSta_enum/1
  Subsystem/5(FGSChCmd) -> VTHC_FDCFGSChCmd_enum/1
  Subsystem/6(FDC_FGS_IONSW_Sta) -> VTHC_FDCFGSIONSWSta_flg/1
  Subsystem/7(FDC_FGS_ION_Cmd) -> VTHC_FDCFGSIONCmd_flg/1
  VINP_IVIZon1WindDirSWReqSta_flg/1 -> Detect Increase7/1
  Detect Increase7/1 -> Logical Operator20/2
  Logical Operator20/1 -> [WindDirP]
  Constant79/1 -> Chart/93(KTHC_ScreenUniq_flg)
  [UserNow] -> Detect Change1/1
  Chart/20(Loading) -> [Loading]
  Chart/4(sigAirIntenZon1St) -> Subsystem1/2(DataIn)
  [Loading] -> Subsystem1/1(Load)
  [Loading] -> Subsystem2/1(Load)
  [Loading] -> Subsystem3/1(Load)
  Chart/2(CCU_ACMaxLampSts) -> Subsystem3/2(DataIn)  "VTHC_CCUACMaxLampSts_flg"
  Chart/6(CCU_AutoLampSts) -> Subsystem4/2(DataIn)  "VTHC_CCUAutoLampSts_flg"
  [Loading] -> Subsystem4/1(Load)
  [Loading] -> Subsystem5/1(Load)
  Chart/1(CCU_ACLampSts) -> Subsystem5/2(DataIn)
  Chart/5(sigWindDirZon1St) -> Subsystem6/2(DataIn)  "VTHC_sigWindDirZon1St_enum"
  [Loading] -> Subsystem6/1(Load)
  [sigRecircSt] -> Subsystem7/2(DataIn)  "VTHC_sigRecircSt_flg"
  [Loading] -> Subsystem7/1(Load)
  [Loading] -> Subsystem8/1(Load)
  Subsystem8/1(DataOut) -> Frost/1  "VTHC_Frost_flg"
  Subsystem9/1(DataOut) -> FD_RecyAuto_Cmd/1  "FD_RecyAuto_Cmd"
  [Loading] -> Subsystem9/1(Load)
  Subsystem10/1(DataOut) -> ACModeMem/1  "ACModeMem"
  [Loading] -> Subsystem10/1(Load)
  Subsystem11/1(DataOut) -> FaceM/1
  [Loading] -> Subsystem11/1(Load)
  Subsystem12/1(DataOut) -> FootM/1
  [Loading] -> Subsystem12/1(Load)
  [Loading] -> Subsystem13/1(Load)
  [Loading] -> Subsystem14/1(Load)
  Chart/17(fdefog) -> [fdefog]  "VTHC_sigDfrstSt_flg"
  [Loading] -> Subsystem15/1(Load)
  [RecyAutoFlg] -> Subsystem16/2(DataIn)
  [Loading] -> Subsystem16/1(Load)
  [Loading] -> Subsystem17/1(Load)
  VBCM_UserNow_enum/1 -> [UserNow]
  [UserNow] -> VALUE_TYPE_ACModeMem/1(UserNow)
  Constant80/1 -> Data Type Conversion13/1
  Data Type Conversion13/1 -> Unit Delay3/1
  Unit Delay3/1 -> Unit Delay11/1
  Unit Delay11/1 -> Unit Delay2/1, [Loadbar]
  [Loadbar] -> VALUE_TYPE_ACModeMem/2(Loadbar)
  VINP_UpdateReq_enum/1 -> [UpdateReq]
  [UpdateReq] -> VALUE_TYPE_ACModeMem/3(UpdateReq)
  Constant81/1 -> Data Type Conversion14/1
  Data Type Conversion14/1 -> VALUE_TYPE_ACModeMem/7(Default)
  EEP_ACModeSet123/1 -> VALUE_TYPE_ACModeMem/4(EEP_Set123)
  [ACMode] -> Unit Delay12/1
  Unit Delay12/1 -> VALUE_TYPE_ACModeMem/6(SettingIn)
  VALUE_TYPE_ACModeMem/1(Setting) -> [EEP_ACMode]  "EEP_ACMode"
  [EEP_ACMode] -> Data Type Conversion6/1
  VALUE_TYPE_ACModeMem/2(Set123) -> ACModeSet123/1
  [UserNow] -> TOGGLE_TYPE_FACE/1(UserNow)
  [Loadbar] -> TOGGLE_TYPE_FACE/2(Loadbar)
  [UpdateReq] -> TOGGLE_TYPE_FACE/3(UpdateReq)
  [Face] -> Unit Delay13/1
  TOGGLE_TYPE_FACE/1(Setting) -> [EEP_FACE]
  EEP_FACESet/1 -> TOGGLE_TYPE_FACE/5(EEP_Set)
  Data Type Conversion15/1 -> TOGGLE_TYPE_FACE/6(Default)
  Constant82/1 -> Data Type Conversion15/1
  Unit Delay13/1 -> TOGGLE_TYPE_FACE/4(SettingIN)
  TOGGLE_TYPE_FACE/2(Set) -> FACESet/1
  TOGGLE_TYPE_FOOT/2(Set) -> FOOTSet/1
  Unit Delay14/1 -> TOGGLE_TYPE_FOOT/4(SettingIN)
  Constant83/1 -> Data Type Conversion16/1
  Data Type Conversion16/1 -> TOGGLE_TYPE_FOOT/6(Default)
  EEP_FOOTSet/1 -> TOGGLE_TYPE_FOOT/5(EEP_Set)
  TOGGLE_TYPE_FOOT/1(Setting) -> [EEP_FOOT]
  [Foot] -> Unit Delay14/1
  [UpdateReq] -> TOGGLE_TYPE_FOOT/3(UpdateReq)
  [Loadbar] -> TOGGLE_TYPE_FOOT/2(Loadbar)
  [UserNow] -> TOGGLE_TYPE_FOOT/1(UserNow)
  [UserNow] -> TOGGLE_TYPE_FROST/1(UserNow)
  [Loadbar] -> TOGGLE_TYPE_FROST/2(Loadbar)
  [UpdateReq] -> TOGGLE_TYPE_FROST/3(UpdateReq)
  [Frost] -> Unit Delay15/1
  TOGGLE_TYPE_FROST/1(Setting) -> [EEP_Frost]
  EEP_FrostSet/1 -> TOGGLE_TYPE_FROST/5(EEP_Set)
  Data Type Conversion17/1 -> TOGGLE_TYPE_FROST/6(Default)
  Constant84/1 -> Data Type Conversion17/1
  Unit Delay15/1 -> TOGGLE_TYPE_FROST/4(SettingIN)
  TOGGLE_TYPE_FROST/2(Set) -> FrostSet/1
  TOGGLE_TYPE_FACEM/2(Set) -> FaceMSet/1
  Unit Delay16/1 -> TOGGLE_TYPE_FACEM/4(SettingIN)
  Constant85/1 -> Data Type Conversion18/1
  Data Type Conversion18/1 -> TOGGLE_TYPE_FACEM/6(Default)
  EEP_FaceMSet/1 -> TOGGLE_TYPE_FACEM/5(EEP_Set)
  TOGGLE_TYPE_FACEM/1(Setting) -> [EEP_FaceM]
  [FaceM] -> Unit Delay16/1
  [UpdateReq] -> TOGGLE_TYPE_FACEM/3(UpdateReq)
  [Loadbar] -> TOGGLE_TYPE_FACEM/2(Loadbar)
  [UserNow] -> TOGGLE_TYPE_FACEM/1(UserNow)
  [UserNow] -> TOGGLE_TYPE_FOOTM/1(UserNow)
  [Loadbar] -> TOGGLE_TYPE_FOOTM/2(Loadbar)
  [UpdateReq] -> TOGGLE_TYPE_FOOTM/3(UpdateReq)
  [FootM] -> Unit Delay17/1
  TOGGLE_TYPE_FOOTM/1(Setting) -> [EEP_FootM]
  EEP_FootMSet/1 -> TOGGLE_TYPE_FOOTM/5(EEP_Set)
  Data Type Conversion19/1 -> TOGGLE_TYPE_FOOTM/6(Default)
  Constant86/1 -> Data Type Conversion19/1
  Unit Delay17/1 -> TOGGLE_TYPE_FOOTM/4(SettingIN)
  TOGGLE_TYPE_FOOTM/2(Set) -> FootMSet/1
  TOGGLE_TYPE_fdefog/2(Set) -> fdefogSet/1
  Unit Delay18/1 -> TOGGLE_TYPE_fdefog/4(SettingIN)
  Constant87/1 -> Data Type Conversion20/1
  Data Type Conversion20/1 -> TOGGLE_TYPE_fdefog/6(Default)
  EEP_fdefogSet/1 -> TOGGLE_TYPE_fdefog/5(EEP_Set)
  TOGGLE_TYPE_fdefog/1(Setting) -> [EEP_fdefog]
  [fdefog] -> Unit Delay18/1
  [UpdateReq] -> TOGGLE_TYPE_fdefog/3(UpdateReq)
  [Loadbar] -> TOGGLE_TYPE_fdefog/2(Loadbar)
  [UserNow] -> TOGGLE_TYPE_fdefog/1(UserNow)
  [UserNow] -> TOGGLE_TYPE_CCUSyncSts/1(UserNow)
  [Loadbar] -> TOGGLE_TYPE_CCUSyncSts/2(Loadbar)
  [UpdateReq] -> TOGGLE_TYPE_CCUSyncSts/3(UpdateReq)
  [VTHC_CCUSyncSts_flg] -> Unit Delay19/1
  TOGGLE_TYPE_CCUSyncSts/1(Setting) -> [EEP_CCUSyncSts]
  EEP_CCUSyncStsSet/1 -> TOGGLE_TYPE_CCUSyncSts/5(EEP_Set)
  Data Type Conversion21/1 -> TOGGLE_TYPE_CCUSyncSts/6(Default)
  Constant88/1 -> Data Type Conversion21/1
  Unit Delay19/1 -> TOGGLE_TYPE_CCUSyncSts/4(SettingIN)
  TOGGLE_TYPE_CCUSyncSts/2(Set) -> CCUSyncStsSet/1
  TOGGLE_TYPE_sigRecircSt/2(Set) -> sigRecircStSet/1
  Unit Delay20/1 -> TOGGLE_TYPE_sigRecircSt/4(SettingIN)
  Constant89/1 -> Data Type Conversion22/1
  Data Type Conversion22/1 -> TOGGLE_TYPE_sigRecircSt/6(Default)
  EEP_sigRecircStSet/1 -> TOGGLE_TYPE_sigRecircSt/5(EEP_Set)
  TOGGLE_TYPE_sigRecircSt/1(Setting) -> [EEP_sigRecircSt]
  [sigRecircSt] -> Unit Delay20/1
  [UpdateReq] -> TOGGLE_TYPE_sigRecircSt/3(UpdateReq)
  [Loadbar] -> TOGGLE_TYPE_sigRecircSt/2(Loadbar)
  [UserNow] -> TOGGLE_TYPE_sigRecircSt/1(UserNow)
  [UserNow] -> TOGGLE_TYPE_RecyAutoFlg/1(UserNow)
  [Loadbar] -> TOGGLE_TYPE_RecyAutoFlg/2(Loadbar)
  [UpdateReq] -> TOGGLE_TYPE_RecyAutoFlg/3(UpdateReq)
  [RecyAutoFlg] -> Unit Delay21/1
  TOGGLE_TYPE_RecyAutoFlg/1(Setting) -> [EEP_RecyAutoFlg]
  EEP_RecyAutoSet/1 -> TOGGLE_TYPE_RecyAutoFlg/5(EEP_Set)
  Data Type Conversion23/1 -> TOGGLE_TYPE_RecyAutoFlg/6(Default)
  Constant90/1 -> Data Type Conversion23/1
  Unit Delay21/1 -> TOGGLE_TYPE_RecyAutoFlg/4(SettingIN)
  TOGGLE_TYPE_RecyAutoFlg/2(Set) -> RecyAutoSet/1
  Subsystem17/1(DataOut) -> AirIntenZone1M/1
  [AirIntenZone1M] -> Unit Delay22/1
  Unit Delay22/1 -> VALUE_TYPE_AirIntenZone1M/4(SettingIN)
  [UserNow] -> VALUE_TYPE_AirIntenZone1M/1(UserNow)
  [Loadbar] -> VALUE_TYPE_AirIntenZone1M/2(Loadbar)
  [UpdateReq] -> VALUE_TYPE_AirIntenZone1M/3(UpdateReq)
  EEP_AirIntenZone1MSet1/1 -> VALUE_TYPE_AirIntenZone1M/5(EEP_Set1)
  EEP_AirIntenZone1MSet2/1 -> VALUE_TYPE_AirIntenZone1M/6(EEP_Set2)
  EEP_AirIntenZone1MSet3/1 -> VALUE_TYPE_AirIntenZone1M/7(EEP_Set3)
  EEP_AirIntenZone1MSet4/1 -> VALUE_TYPE_AirIntenZone1M/8(EEP_Set4)
  EEP_AirIntenZone1MSet5/1 -> VALUE_TYPE_AirIntenZone1M/9(EEP_Set5)
  EEP_AirIntenZone1MSet7/1 -> VALUE_TYPE_AirIntenZone1M/10(EEP_Set7)
  Data Type Conversion24/1 -> VALUE_TYPE_AirIntenZone1M/11(Default)
  Constant91/1 -> Data Type Conversion24/1
  VALUE_TYPE_AirIntenZone1M/1(Setting) -> [EEP_AirIntenZone1M]
  VALUE_TYPE_AirIntenZone1M/2(Set1) -> AirIntenZone1MSet1/1
  VALUE_TYPE_AirIntenZone1M/7(Set7) -> AirIntenZone1MSet7/1
  VALUE_TYPE_AirIntenZone1M/6(Set5) -> AirIntenZone1MSet5/1
  VALUE_TYPE_AirIntenZone1M/5(Set4) -> AirIntenZone1MSet4/1
  VALUE_TYPE_AirIntenZone1M/4(Set3) -> AirIntenZone1MSet3/1
  VALUE_TYPE_AirIntenZone1M/3(Set2) -> AirIntenZone1MSet2/1
  [Loading] -> Subsystem18/1(Load)
  Switch24/1 -> Subsystem18/2(DataIn)
  Logical Operator21/1 -> Switch24/2
  [fInitial] -> Logical Operator9/1
  [Loading] -> Logical Operator21/2
  VALUE_TYPE_AirIntenZone3M/3(Set2) -> AirIntenZone3MSet2/1
  VALUE_TYPE_AirIntenZone3M/4(Set3) -> AirIntenZone3MSet3/1
  VALUE_TYPE_AirIntenZone3M/5(Set4) -> AirIntenZone3MSet4/1
  VALUE_TYPE_AirIntenZone3M/6(Set5) -> AirIntenZone3MSet5/1
  VALUE_TYPE_AirIntenZone3M/7(Set7) -> AirIntenZone3MSet7/1
  VALUE_TYPE_AirIntenZone3M/2(Set1) -> AirIntenZone3MSet1/1
  VALUE_TYPE_AirIntenZone3M/1(Setting) -> [EEP_AirIntenZone3M]
  Constant92/1 -> Data Type Conversion25/1
  Data Type Conversion25/1 -> VALUE_TYPE_AirIntenZone3M/11(Default)
  EEP_AirIntenZone3MSet7/1 -> VALUE_TYPE_AirIntenZone3M/10(EEP_Set7)
  EEP_AirIntenZone3MSet5/1 -> VALUE_TYPE_AirIntenZone3M/9(EEP_Set5)
  EEP_AirIntenZone3MSet4/1 -> VALUE_TYPE_AirIntenZone3M/8(EEP_Set4)
  EEP_AirIntenZone3MSet3/1 -> VALUE_TYPE_AirIntenZone3M/7(EEP_Set3)
  EEP_AirIntenZone3MSet2/1 -> VALUE_TYPE_AirIntenZone3M/6(EEP_Set2)
  EEP_AirIntenZone3MSet1/1 -> VALUE_TYPE_AirIntenZone3M/5(EEP_Set1)
  [UpdateReq] -> VALUE_TYPE_AirIntenZone3M/3(UpdateReq)
  [Loadbar] -> VALUE_TYPE_AirIntenZone3M/2(Loadbar)
  [UserNow] -> VALUE_TYPE_AirIntenZone3M/1(UserNow)
  Unit Delay23/1 -> VALUE_TYPE_AirIntenZone3M/4(SettingIN)
  [AirIntenZone3M] -> Unit Delay23/1
  [UserNow] -> TOGGLE_TYPE_IONSWSta/1(UserNow)
  [Loadbar] -> TOGGLE_TYPE_IONSWSta/2(Loadbar)
  [UpdateReq] -> TOGGLE_TYPE_IONSWSta/3(UpdateReq)
  VINP_IVIIONSWCmd_flg/1 -> TOGGLE_TYPE_IONSWSta/4(iviCMD)
  EEP_IONSWStaSet/1 -> TOGGLE_TYPE_IONSWSta/5(EEP_Set)
  Data Type Conversion26/1 -> TOGGLE_TYPE_IONSWSta/6(Default)
  Constant93/1 -> Data Type Conversion26/1
  TOGGLE_TYPE_IONSWSta/1(Setting) -> [EEP_IONSWSta]
  TOGGLE_TYPE_IONSWSta/2(Set) -> IONSWStaSet/1
  [EEP_IONSWSta] -> Subsystem/4(EEP_IONSWSta)
  VALUE_TYPE_FDCFGSChStaSet/2(Set123) -> FDCFGSChStaSet123/1
  EEP_FDCFGSChStaSet123/1 -> VALUE_TYPE_FDCFGSChStaSet/4(EEP_Set123)
  Data Type Conversion27/1 -> VALUE_TYPE_FDCFGSChStaSet/7(Default)
  Constant94/1 -> Data Type Conversion27/1
  [UpdateReq] -> VALUE_TYPE_FDCFGSChStaSet/3(UpdateReq)
  [Loadbar] -> VALUE_TYPE_FDCFGSChStaSet/2(Loadbar)
  [UserNow] -> VALUE_TYPE_FDCFGSChStaSet/1(UserNow)
  VINP_IVIFGSChCmd_enum/1 -> VALUE_TYPE_FDCFGSChStaSet/6(SettingIn)
  [EEP_FDCFGSChSta] -> Subsystem/2(EEP_FDCFGSChSta)
  [UserNow] -> VALUE_TYPE_FDCFGSAirIntSta/1(UserNow)
  [Loadbar] -> VALUE_TYPE_FDCFGSAirIntSta/2(Loadbar)
  [UpdateReq] -> VALUE_TYPE_FDCFGSAirIntSta/3(UpdateReq)
  Constant95/1 -> Data Type Conversion28/1
  Data Type Conversion28/1 -> VALUE_TYPE_FDCFGSAirIntSta/7(Default)
  EEP_FDCFGSAirIntStaSet123/1 -> VALUE_TYPE_FDCFGSAirIntSta/4(EEP_Set123)
  VALUE_TYPE_FDCFGSAirIntSta/2(Set123) -> FDCFGSAirIntStaSet123/1
  [EEP_FDCFGSAirIntSta] -> Subsystem/1(EEP_FDCFGSAirIntSta)
  [Loading] -> Subsystem19/1(Load)
  [Loading] -> Subsystem20/1(Load)
  [Loading] -> Subsystem21/1(Load)
  [Loading] -> Subsystem22/1(Load)
  [Loading] -> Subsystem23/1(Load)
  [Loading] -> Subsystem24/1(Load)
  [Loading] -> Subsystem25/1(Load)
  [Loading] -> Subsystem26/1(Load)
  [Loading] -> Subsystem27/1(Load)
  [Loading] -> Subsystem28/1(Load)
  [Loading] -> Subsystem29/1(Load)
  [Loading] -> Subsystem30/1(Load)
  [Loading] -> Subsystem31/1(Load)
  [Loading] -> Subsystem32/1(Load)
  [UserNow] -> TOGGLE_TYPE_LVentEN/1(UserNow)
  [Loadbar] -> TOGGLE_TYPE_LVentEN/2(Loadbar)
  [UpdateReq] -> TOGGLE_TYPE_LVentEN/3(UpdateReq)
  Unit Delay24/1 -> TOGGLE_TYPE_LVentEN/4(SettingIN)
  [LVentEN] -> Unit Delay24/1
  TOGGLE_TYPE_LVentEN/1(Setting) -> [EEP_LVentEN]
  TOGGLE_TYPE_LVentEN/2(Set) -> LVentENSet/1
  EEP_LVentENSet/1 -> TOGGLE_TYPE_LVentEN/5(EEP_Set)
  Data Type Conversion29/1 -> TOGGLE_TYPE_LVentEN/6(Default)
  Constant96/1 -> Data Type Conversion29/1
  Constant97/1 -> Data Type Conversion30/1
  Data Type Conversion30/1 -> TOGGLE_TYPE_CLVentEN/6(Default)
  EEP_CLVentENSet/1 -> TOGGLE_TYPE_CLVentEN/5(EEP_Set)
  TOGGLE_TYPE_CLVentEN/2(Set) -> CLVentENSet/1
  TOGGLE_TYPE_CLVentEN/1(Setting) -> [EEP_CLVentEN]
  [CLVentEN] -> Unit Delay25/1
  Unit Delay25/1 -> TOGGLE_TYPE_CLVentEN/4(SettingIN)
  [UpdateReq] -> TOGGLE_TYPE_CLVentEN/3(UpdateReq)
  [Loadbar] -> TOGGLE_TYPE_CLVentEN/2(Loadbar)
  [UserNow] -> TOGGLE_TYPE_CLVentEN/1(UserNow)
  [UserNow] -> TOGGLE_TYPE_RVentEN/1(UserNow)
  [Loadbar] -> TOGGLE_TYPE_RVentEN/2(Loadbar)
  [UpdateReq] -> TOGGLE_TYPE_RVentEN/3(UpdateReq)
  Unit Delay26/1 -> TOGGLE_TYPE_RVentEN/4(SettingIN)
  [RVentEN] -> Unit Delay26/1
  TOGGLE_TYPE_RVentEN/1(Setting) -> [EEP_RVentEN]
  TOGGLE_TYPE_RVentEN/2(Set) -> RVentENSet/1
  EEP_RVentENSet/1 -> TOGGLE_TYPE_RVentEN/5(EEP_Set)
  Data Type Conversion31/1 -> TOGGLE_TYPE_RVentEN/6(Default)
  Constant98/1 -> Data Type Conversion31/1
  Constant99/1 -> Data Type Conversion32/1
  Data Type Conversion32/1 -> TOGGLE_TYPE_CRVentEN/6(Default)
  EEP_CRVentENSet/1 -> TOGGLE_TYPE_CRVentEN/5(EEP_Set)
  TOGGLE_TYPE_CRVentEN/2(Set) -> CRVentENSet/1
  TOGGLE_TYPE_CRVentEN/1(Setting) -> [EEP_CRVentEN]
  [CRVentEN] -> Unit Delay27/1
  Unit Delay27/1 -> TOGGLE_TYPE_CRVentEN/4(SettingIN)
  [UpdateReq] -> TOGGLE_TYPE_CRVentEN/3(UpdateReq)
  [Loadbar] -> TOGGLE_TYPE_CRVentEN/2(Loadbar)
  [UserNow] -> TOGGLE_TYPE_CRVentEN/1(UserNow)
  VALUE_TYPE_LEventModeSta/2(Set123) -> FDCTHCLEventModeStaSet123/1
  VALUE_TYPE_LEventModeSta/1(Setting) -> [EEP_FDCTHCLEventModeSta]
  Unit Delay28/1 -> VALUE_TYPE_LEventModeSta/6(SettingIn)
  [FDCTHCLEventModeSta] -> Unit Delay28/1
  EEP_FDCTHCLEventModeStaSet123/1 -> VALUE_TYPE_LEventModeSta/4(EEP_Set123)
  Data Type Conversion33/1 -> VALUE_TYPE_LEventModeSta/7(Default)
  Constant100/1 -> Data Type Conversion33/1
  [UpdateReq] -> VALUE_TYPE_LEventModeSta/3(UpdateReq)
  [Loadbar] -> VALUE_TYPE_LEventModeSta/2(Loadbar)
  [UserNow] -> VALUE_TYPE_LEventModeSta/1(UserNow)
  [UserNow] -> VALUE_TYPE_REventModeSta/1(UserNow)
  [Loadbar] -> VALUE_TYPE_REventModeSta/2(Loadbar)
  [UpdateReq] -> VALUE_TYPE_REventModeSta/3(UpdateReq)
  Constant101/1 -> Data Type Conversion34/1
  Data Type Conversion34/1 -> VALUE_TYPE_REventModeSta/7(Default)
  EEP_FDCTHCREventModeStaSet123/1 -> VALUE_TYPE_REventModeSta/4(EEP_Set123)
  [FDCTHCREventModeSta] -> Unit Delay29/1
  Unit Delay29/1 -> VALUE_TYPE_REventModeSta/6(SettingIn)
  VALUE_TYPE_REventModeSta/1(Setting) -> [EEP_FDCTHCREventModeSta]
  VALUE_TYPE_REventModeSta/2(Set123) -> FDCTHCREventModeStaSet123/1
  [EEP_FDCTHCLEventModeSta] -> EVent/3(VINP_FDCTHCLEventModeStaM_enum)
  [EEP_FDCTHCREventModeSta] -> EVent/5(VINP_FDCTHCREventModeStaM_enum)
  VALUE_TYPE_FDCTHCREventZSta/3(Set2) -> FDCTHCREventZStaSet2/1
  Constant103/1 -> Data Type Conversion36/1
  Unit Delay30/1 -> VALUE_TYPE_FDCTHCCLEVentZSta/4(SettingIN)
  [UpdateReq] -> VALUE_TYPE_FDCTHCCLEVentZSta/3(UpdateReq)
  EEP_FDCTHCCLEVentZStaSet5/1 -> VALUE_TYPE_FDCTHCCLEVentZSta/9(EEP_Set5)
  EEP_FDCTHCCLEVentZStaSet3/1 -> VALUE_TYPE_FDCTHCCLEVentZSta/7(EEP_Set3)
  VALUE_TYPE_FDCTHCCLEVentZSta/5(Set4) -> FDCTHCCLEVentZStaSet4/1
  VALUE_TYPE_FDCTHCCLEVentZSta/3(Set2) -> FDCTHCCLEVentZStaSet2/1
  Constant102/1 -> Data Type Conversion35/1
  VALUE_TYPE_FDCTHCCLEVentZSta/2(Set1) -> FDCTHCCLEVentZStaSet1/1
  VALUE_TYPE_FDCTHCCLEVentZSta/7(Set7) -> FDCTHCCLEVentZStaSet7/1
  [UpdateReq] -> VALUE_TYPE_FDCTHCLEventZSta/3(UpdateReq)
  Data Type Conversion36/1 -> VALUE_TYPE_FDCTHCREventZSta/11(Default)
  VALUE_TYPE_FDCTHCREventZSta/1(Setting) -> [EEP_FDCTHCREventZSta]
  VALUE_TYPE_FDCTHCREventZSta/6(Set5) -> FDCTHCREventZStaSet5/1
  EEP_FDCTHCREventZStaSet1/1 -> VALUE_TYPE_FDCTHCREventZSta/5(EEP_Set1)
  Unit Delay31/1 -> VALUE_TYPE_FDCTHCREventZSta/4(SettingIN)
  EEP_FDCTHCREventZStaSet2/1 -> VALUE_TYPE_FDCTHCREventZSta/6(EEP_Set2)
  EEP_FDCTHCREventZStaSet7/1 -> VALUE_TYPE_FDCTHCREventZSta/10(EEP_Set7)
  VALUE_TYPE_FDCTHCREventZSta/2(Set1) -> FDCTHCREventZStaSet1/1
  EEP_FDCTHCREventZStaSet4/1 -> VALUE_TYPE_FDCTHCREventZSta/8(EEP_Set4)
  VALUE_TYPE_FDCTHCCLEVentZSta/6(Set5) -> FDCTHCCLEVentZStaSet5/1
  VALUE_TYPE_FDCTHCCLEVentZSta/1(Setting) -> [EEP_FDCTHCCLEVentZSta]
  [UpdateReq] -> VALUE_TYPE_FDCTHCCREVentZSta/3(UpdateReq)
  EEP_FDCTHCCLEVentZStaSet4/1 -> VALUE_TYPE_FDCTHCCLEVentZSta/8(EEP_Set4)
  VALUE_TYPE_FDCTHCCREVentZSta/5(Set4) -> FDCTHCCREVentZStaSet4/1
  VALUE_TYPE_FDCTHCCREVentZSta/3(Set2) -> FDCTHCCREVentZStaSet2/1
  EEP_FDCTHCCLEVentZStaSet2/1 -> VALUE_TYPE_FDCTHCCLEVentZSta/6(EEP_Set2)
  Constant104/1 -> Data Type Conversion38/1
  VALUE_TYPE_FDCTHCCREVentZSta/2(Set1) -> FDCTHCCREVentZStaSet1/1
  Data Type Conversion37/1 -> VALUE_TYPE_FDCTHCLEventZSta/11(Default)
  VALUE_TYPE_FDCTHCLEventZSta/3(Set2) -> FDCTHCLEventZStaSet2/1
  VALUE_TYPE_FDCTHCCREVentZSta/7(Set7) -> FDCTHCCREVentZStaSet7/1
  Constant105/1 -> Data Type Conversion37/1
  VALUE_TYPE_FDCTHCLEventZSta/5(Set4) -> FDCTHCLEventZStaSet4/1
  VALUE_TYPE_FDCTHCLEventZSta/7(Set7) -> FDCTHCLEventZStaSet7/1
  EEP_FDCTHCCREVentZStaSet5/1 -> VALUE_TYPE_FDCTHCCREVentZSta/9(EEP_Set5)
  EEP_FDCTHCLEventZStaSet7/1 -> VALUE_TYPE_FDCTHCLEventZSta/10(EEP_Set7)
  EEP_FDCTHCCLEVentZStaSet7/1 -> VALUE_TYPE_FDCTHCCLEVentZSta/10(EEP_Set7)
  VALUE_TYPE_FDCTHCCLEVentZSta/4(Set3) -> FDCTHCCLEVentZStaSet3/1
  [FDCTHCCLEVentZSta] -> Unit Delay30/1
  [FDCTHCLEventZSta] -> Unit Delay32/1
  VALUE_TYPE_FDCTHCREventZSta/5(Set4) -> FDCTHCREventZStaSet4/1
  [UserNow] -> VALUE_TYPE_FDCTHCCREVentZSta/1(UserNow)
  VALUE_TYPE_FDCTHCREventZSta/4(Set3) -> FDCTHCREventZStaSet3/1
  EEP_FDCTHCREventZStaSet5/1 -> VALUE_TYPE_FDCTHCREventZSta/9(EEP_Set5)
  VALUE_TYPE_FDCTHCCREVentZSta/4(Set3) -> FDCTHCCREVentZStaSet3/1
  Data Type Conversion38/1 -> VALUE_TYPE_FDCTHCCREVentZSta/11(Default)
  EEP_FDCTHCCLEVentZStaSet1/1 -> VALUE_TYPE_FDCTHCCLEVentZSta/5(EEP_Set1)
  [Loadbar] -> VALUE_TYPE_FDCTHCREventZSta/2(Loadbar)
  [Loadbar] -> VALUE_TYPE_FDCTHCLEventZSta/2(Loadbar)
  Data Type Conversion35/1 -> VALUE_TYPE_FDCTHCCLEVentZSta/11(Default)
  VALUE_TYPE_FDCTHCLEventZSta/6(Set5) -> FDCTHCLEventZStaSet5/1
  EEP_FDCTHCLEventZStaSet3/1 -> VALUE_TYPE_FDCTHCLEventZSta/7(EEP_Set3)
  EEP_FDCTHCLEventZStaSet1/1 -> VALUE_TYPE_FDCTHCLEventZSta/5(EEP_Set1)
  EEP_FDCTHCCREVentZStaSet4/1 -> VALUE_TYPE_FDCTHCCREVentZSta/8(EEP_Set4)
  [Loadbar] -> VALUE_TYPE_FDCTHCCLEVentZSta/2(Loadbar)
  [FDCTHCCREVentZSta] -> Unit Delay33/1
  EEP_FDCTHCCREVentZStaSet1/1 -> VALUE_TYPE_FDCTHCCREVentZSta/5(EEP_Set1)
  EEP_FDCTHCCREVentZStaSet7/1 -> VALUE_TYPE_FDCTHCCREVentZSta/10(EEP_Set7)
  EEP_FDCTHCLEventZStaSet5/1 -> VALUE_TYPE_FDCTHCLEventZSta/9(EEP_Set5)
  EEP_FDCTHCREventZStaSet3/1 -> VALUE_TYPE_FDCTHCREventZSta/7(EEP_Set3)
  [UserNow] -> VALUE_TYPE_FDCTHCCLEVentZSta/1(UserNow)
  EEP_FDCTHCCREVentZStaSet3/1 -> VALUE_TYPE_FDCTHCCREVentZSta/7(EEP_Set3)
  Unit Delay33/1 -> VALUE_TYPE_FDCTHCCREVentZSta/4(SettingIN)
  EEP_FDCTHCLEventZStaSet2/1 -> VALUE_TYPE_FDCTHCLEventZSta/6(EEP_Set2)
  VALUE_TYPE_FDCTHCREventZSta/7(Set7) -> FDCTHCREventZStaSet7/1
  [UpdateReq] -> VALUE_TYPE_FDCTHCREventZSta/3(UpdateReq)
  VALUE_TYPE_FDCTHCLEventZSta/1(Setting) -> [EEP_FDCTHCLEventZSta]
  [UserNow] -> VALUE_TYPE_FDCTHCREventZSta/1(UserNow)
  EEP_FDCTHCCREVentZStaSet2/1 -> VALUE_TYPE_FDCTHCCREVentZSta/6(EEP_Set2)
  VALUE_TYPE_FDCTHCCREVentZSta/6(Set5) -> FDCTHCCREVentZStaSet5/1
  VALUE_TYPE_FDCTHCLEventZSta/2(Set1) -> FDCTHCLEventZStaSet1/1
  Unit Delay32/1 -> VALUE_TYPE_FDCTHCLEventZSta/4(SettingIN)
  [Loadbar] -> VALUE_TYPE_FDCTHCCREVentZSta/2(Loadbar)
  VALUE_TYPE_FDCTHCCREVentZSta/1(Setting) -> [EEP_FDCTHCCREVentZSta]
  [UserNow] -> VALUE_TYPE_FDCTHCLEventZSta/1(UserNow)
  [FDCTHCREventZSta] -> Unit Delay31/1
  VALUE_TYPE_FDCTHCLEventZSta/4(Set3) -> FDCTHCLEventZStaSet3/1
  EEP_FDCTHCLEventZStaSet4/1 -> VALUE_TYPE_FDCTHCLEventZSta/8(EEP_Set4)
  VALUE_TYPE_FDCTHCREventYSta/3(Set2) -> FDCTHCREventYStaSet2/1
  Constant107/1 -> Data Type Conversion40/1
  Unit Delay34/1 -> VALUE_TYPE_FDCTHCCLEVentYSta/4(SettingIN)
  [UpdateReq] -> VALUE_TYPE_FDCTHCCLEVentYSta/3(UpdateReq)
  EEP_FDCTHCCLEVentYStaSet5/1 -> VALUE_TYPE_FDCTHCCLEVentYSta/9(EEP_Set5)
  EEP_FDCTHCCLEVentYStaSet3/1 -> VALUE_TYPE_FDCTHCCLEVentYSta/7(EEP_Set3)
  VALUE_TYPE_FDCTHCCLEVentYSta/5(Set4) -> FDCTHCCLEVentYStaSet4/1
  VALUE_TYPE_FDCTHCCLEVentYSta/3(Set2) -> FDCTHCCLEVentYStaSet2/1
  Constant106/1 -> Data Type Conversion39/1
  VALUE_TYPE_FDCTHCCLEVentYSta/2(Set1) -> FDCTHCCLEVentYStaSet1/1
  VALUE_TYPE_FDCTHCCLEVentYSta/7(Set7) -> FDCTHCCLEVentYStaSet7/1
  [UpdateReq] -> VALUE_TYPE_FDCTHCLEventYSta/3(UpdateReq)
  Data Type Conversion40/1 -> VALUE_TYPE_FDCTHCREventYSta/11(Default)
  VALUE_TYPE_FDCTHCREventYSta/1(Setting) -> [EEP_FDCTHCREventYSta]
  VALUE_TYPE_FDCTHCREventYSta/6(Set5) -> FDCTHCREventYStaSet5/1
  EEP_FDCTHCREventYStaSet1/1 -> VALUE_TYPE_FDCTHCREventYSta/5(EEP_Set1)
  Unit Delay35/1 -> VALUE_TYPE_FDCTHCREventYSta/4(SettingIN)
  EEP_FDCTHCREventYStaSet2/1 -> VALUE_TYPE_FDCTHCREventYSta/6(EEP_Set2)
  EEP_FDCTHCREventYStaSet7/1 -> VALUE_TYPE_FDCTHCREventYSta/10(EEP_Set7)
  VALUE_TYPE_FDCTHCREventYSta/2(Set1) -> FDCTHCREventYStaSet1/1
  EEP_FDCTHCREventYStaSet4/1 -> VALUE_TYPE_FDCTHCREventYSta/8(EEP_Set4)
  VALUE_TYPE_FDCTHCCLEVentYSta/6(Set5) -> FDCTHCCLEVentYStaSet5/1
  VALUE_TYPE_FDCTHCCLEVentYSta/1(Setting) -> [EEP_FDCTHCCLEVentYSta]
  [UpdateReq] -> VALUE_TYPE_FDCTHCCREVentYSta/3(UpdateReq)
  EEP_FDCTHCCLEVentYStaSet4/1 -> VALUE_TYPE_FDCTHCCLEVentYSta/8(EEP_Set4)
  VALUE_TYPE_FDCTHCCREVentYSta/5(Set4) -> FDCTHCCREVentYStaSet4/1
  VALUE_TYPE_FDCTHCCREVentYSta/3(Set2) -> FDCTHCCREVentYStaSet2/1
  EEP_FDCTHCCLEVentYStaSet2/1 -> VALUE_TYPE_FDCTHCCLEVentYSta/6(EEP_Set2)
  Constant108/1 -> Data Type Conversion42/1
  VALUE_TYPE_FDCTHCCREVentYSta/2(Set1) -> FDCTHCCREVentYStaSet1/1
  Data Type Conversion41/1 -> VALUE_TYPE_FDCTHCLEventYSta/11(Default)
  VALUE_TYPE_FDCTHCLEventYSta/3(Set2) -> FDCTHCLEventYStaSet2/1
  VALUE_TYPE_FDCTHCCREVentYSta/7(Set7) -> FDCTHCCREVentYStaSet7/1
  Constant109/1 -> Data Type Conversion41/1
  VALUE_TYPE_FDCTHCLEventYSta/5(Set4) -> FDCTHCLEventYStaSet4/1
  VALUE_TYPE_FDCTHCLEventYSta/7(Set7) -> FDCTHCLEventYStaSet7/1
  EEP_FDCTHCCREVentYStaSet5/1 -> VALUE_TYPE_FDCTHCCREVentYSta/9(EEP_Set5)
  EEP_FDCTHCLEventYStaSet7/1 -> VALUE_TYPE_FDCTHCLEventYSta/10(EEP_Set7)
  EEP_FDCTHCCLEVentYStaSet7/1 -> VALUE_TYPE_FDCTHCCLEVentYSta/10(EEP_Set7)
  VALUE_TYPE_FDCTHCCLEVentYSta/4(Set3) -> FDCTHCCLEVentYStaSet3/1
  [FDCTHCCLEVentYSta] -> Unit Delay34/1
  [FDCTHCLEventYSta] -> Unit Delay36/1
  VALUE_TYPE_FDCTHCREventYSta/5(Set4) -> FDCTHCREventYStaSet4/1
  [UserNow] -> VALUE_TYPE_FDCTHCCREVentYSta/1(UserNow)
  VALUE_TYPE_FDCTHCREventYSta/4(Set3) -> FDCTHCREventYStaSet3/1
  EEP_FDCTHCREventYStaSet5/1 -> VALUE_TYPE_FDCTHCREventYSta/9(EEP_Set5)
  VALUE_TYPE_FDCTHCCREVentYSta/4(Set3) -> FDCTHCCREVentYStaSet3/1
  Data Type Conversion42/1 -> VALUE_TYPE_FDCTHCCREVentYSta/11(Default)
  EEP_FDCTHCCLEVentYStaSet1/1 -> VALUE_TYPE_FDCTHCCLEVentYSta/5(EEP_Set1)
  [Loadbar] -> VALUE_TYPE_FDCTHCREventYSta/2(Loadbar)
  [Loadbar] -> VALUE_TYPE_FDCTHCLEventYSta/2(Loadbar)
  Data Type Conversion39/1 -> VALUE_TYPE_FDCTHCCLEVentYSta/11(Default)
  VALUE_TYPE_FDCTHCLEventYSta/6(Set5) -> FDCTHCLEventYStaSet5/1
  EEP_FDCTHCLEventYStaSet3/1 -> VALUE_TYPE_FDCTHCLEventYSta/7(EEP_Set3)
  EEP_FDCTHCLEventYStaSet1/1 -> VALUE_TYPE_FDCTHCLEventYSta/5(EEP_Set1)
  EEP_FDCTHCCREVentYStaSet4/1 -> VALUE_TYPE_FDCTHCCREVentYSta/8(EEP_Set4)
  [Loadbar] -> VALUE_TYPE_FDCTHCCLEVentYSta/2(Loadbar)
  [FDCTHCCREVentYSta] -> Unit Delay37/1
  EEP_FDCTHCCREVentYStaSet1/1 -> VALUE_TYPE_FDCTHCCREVentYSta/5(EEP_Set1)
  EEP_FDCTHCCREVentYStaSet7/1 -> VALUE_TYPE_FDCTHCCREVentYSta/10(EEP_Set7)
  EEP_FDCTHCLEventYStaSet5/1 -> VALUE_TYPE_FDCTHCLEventYSta/9(EEP_Set5)
  EEP_FDCTHCREventYStaSet3/1 -> VALUE_TYPE_FDCTHCREventYSta/7(EEP_Set3)
  [UserNow] -> VALUE_TYPE_FDCTHCCLEVentYSta/1(UserNow)
  EEP_FDCTHCCREVentYStaSet3/1 -> VALUE_TYPE_FDCTHCCREVentYSta/7(EEP_Set3)
  Unit Delay37/1 -> VALUE_TYPE_FDCTHCCREVentYSta/4(SettingIN)
  EEP_FDCTHCLEventYStaSet2/1 -> VALUE_TYPE_FDCTHCLEventYSta/6(EEP_Set2)
  VALUE_TYPE_FDCTHCREventYSta/7(Set7) -> FDCTHCREventYStaSet7/1
  [UpdateReq] -> VALUE_TYPE_FDCTHCREventYSta/3(UpdateReq)
  VALUE_TYPE_FDCTHCLEventYSta/1(Setting) -> [EEP_FDCTHCLEventYSta]
  [UserNow] -> VALUE_TYPE_FDCTHCREventYSta/1(UserNow)
  EEP_FDCTHCCREVentYStaSet2/1 -> VALUE_TYPE_FDCTHCCREVentYSta/6(EEP_Set2)
  VALUE_TYPE_FDCTHCCREVentYSta/6(Set5) -> FDCTHCCREVentYStaSet5/1
  VALUE_TYPE_FDCTHCLEventYSta/2(Set1) -> FDCTHCLEventYStaSet1/1
  Unit Delay36/1 -> VALUE_TYPE_FDCTHCLEventYSta/4(SettingIN)
  [Loadbar] -> VALUE_TYPE_FDCTHCCREVentYSta/2(Loadbar)
  VALUE_TYPE_FDCTHCCREVentYSta/1(Setting) -> [EEP_FDCTHCCREVentYSta]
  [UserNow] -> VALUE_TYPE_FDCTHCLEventYSta/1(UserNow)
  [FDCTHCREventYSta] -> Unit Delay35/1
  VALUE_TYPE_FDCTHCLEventYSta/4(Set3) -> FDCTHCLEventYStaSet3/1
  EEP_FDCTHCLEventYStaSet4/1 -> VALUE_TYPE_FDCTHCLEventYSta/8(EEP_Set4)
  Unit Delay2/1 -> [fInitial]
  VALUE_TYPE_ACModeMem/3(Set457) -> ACModeSet457/1
  EEP_ACModeSet457/1 -> VALUE_TYPE_ACModeMem/5(EEP_Set457)
  EEP_FDCFGSChStaSet457/1 -> VALUE_TYPE_FDCFGSChStaSet/5(EEP_Set457)
  VALUE_TYPE_FDCFGSChStaSet/3(Set457) -> FDCFGSChStaSet457/1
  EEP_FDCFGSAirIntStaSet457/1 -> VALUE_TYPE_FDCFGSAirIntSta/5(EEP_Set457)
  VALUE_TYPE_FDCFGSAirIntSta/3(Set457) -> FDCFGSAirIntStaSet457/1
  EEP_FDCTHCLEventModeStaSet457/1 -> VALUE_TYPE_LEventModeSta/5(EEP_Set457)
  VALUE_TYPE_LEventModeSta/3(Set457) -> FDCTHCLEventModeStaSet457/1
  EEP_FDCTHCREventModeStaSet457/1 -> VALUE_TYPE_REventModeSta/5(EEP_Set457)
  VALUE_TYPE_REventModeSta/3(Set457) -> FDCTHCREventModeStaSet457/1
  SettempToRawData/1(RawOut) -> [SettempZon1Raw]
  Switch12/1 -> VTHC_sigSetTempZon2StM_C/1, Unit Delay1/1, Switch/3  "VTHC_sigSetTempZon2StM_C"
  VALUE_TYPE_SettempZon1/3(Set2) -> SettempZon1Set2/1
  VALUE_TYPE_SettempZon1/4(Set3) -> SettempZon1Set3/1
  VALUE_TYPE_SettempZon1/5(Set4) -> SettempZon1Set4/1
  VALUE_TYPE_SettempZon1/6(Set5) -> SettempZon1Set5/1
  VALUE_TYPE_SettempZon1/7(Set7) -> SettempZon1Set7/1
  VALUE_TYPE_SettempZon1/2(Set1) -> SettempZon1Set1/1
  VALUE_TYPE_SettempZon1/1(Setting) -> [EEP_SettempZon1]
  Constant55/1 -> Data Type Conversion43/1
  Data Type Conversion43/1 -> VALUE_TYPE_SettempZon1/11(Default)
  EEP_SettempZon1Set7/1 -> VALUE_TYPE_SettempZon1/10(EEP_Set7)
  EEP_SettempZon1Set5/1 -> VALUE_TYPE_SettempZon1/9(EEP_Set5)
  EEP_SettempZon1Set4/1 -> VALUE_TYPE_SettempZon1/8(EEP_Set4)
  EEP_SettempZon1Set3/1 -> VALUE_TYPE_SettempZon1/7(EEP_Set3)
  EEP_SettempZon1Set2/1 -> VALUE_TYPE_SettempZon1/6(EEP_Set2)
  EEP_SettempZon1Set1/1 -> VALUE_TYPE_SettempZon1/5(EEP_Set1)
  [UpdateReq] -> VALUE_TYPE_SettempZon1/3(UpdateReq)
  [Loadbar] -> VALUE_TYPE_SettempZon1/2(Loadbar)
  [UserNow] -> VALUE_TYPE_SettempZon1/1(UserNow)
  Unit Delay38/1 -> VALUE_TYPE_SettempZon1/4(SettingIN)
  [SettempZon1Raw] -> Unit Delay38/1
  [fInitial] -> Logical Operator26/1
  [Loading] -> Logical Operator23/1
  [EEP_SettempZon1] -> RawdataToSettemp/1(RawIN)
  Data Type Conversion12/1 -> Subsystem33/2(DataIn)  "VTHC_sigSetTempZon1St_C"
  [Loading] -> Subsystem33/1(Load)
  Logical Operator25/1 -> Switch12/2
  Switch/1 -> VTHC_sigSetTempZon2St_C/1, Add8/1, Unit Delay7/1  "VTHC_sigSetTempZon2St_C"
  Logical Operator26/1 -> Logical Operator23/2
  Chart/14(FootM) -> [FootM]
  Chart/3(CCU_SyncSts) -> [VTHC_CCUSyncSts_flg]
  [VTHC_CCUSyncSts_flg] -> Subsystem2/2(DataIn)
  Chart/7(sigRecircSt) -> [sigRecircSt]  "VTHC_sigRecircSt_flg"
  Chart/9(Frost) -> [Frost]
  [WaterFillReq] -> WaterFillReq/1
  Chart/11(FD_RecyAuto_Cmd) -> Subsystem9/2(DataIn)
  [ACMode] -> Subsystem10/2(DataIn)
  [FaceM] -> Subsystem11/2(DataIn)
  [FootM] -> Subsystem12/2(DataIn)
  Chart/15(Face) -> [Face]
  [Face] -> Subsystem13/2(DataIn)
  Chart/16(Foot) -> [Foot]
  [Foot] -> Subsystem14/2(DataIn)
  [fdefog] -> Subsystem15/2(DataIn)
  [AirIntenZone1M] -> Subsystem17/2(DataIn)
  Detect Change1/1 -> Chart/94(UserChange)
  Chart/18(RecAutoFlg) -> [RecyAutoFlg]
  VALUE_TYPE_FDCFGSChStaSet/1(Setting) -> [EEP_FDCFGSChSta]
  VALUE_TYPE_FDCFGSAirIntSta/1(Setting) -> [EEP_FDCFGSAirIntSta]
  EVent/1(VTHC_FDCTHCLEventModeSta_enum) -> [FDCTHCLEventModeSta]
  Subsystem19/1(DataOut) -> VTHC_FDCTHCLEventModeSta_enum/1
  [FDCTHCLEventModeSta] -> Subsystem19/2(DataIn)
  Subsystem20/1(DataOut) -> VTHC_FDCTHCREventModeSta_enum/1
  [FDCTHCREventModeSta] -> Subsystem20/2(DataIn)
  EVent/2(VTHC_FDCTHCREventModeSta_enum) -> [FDCTHCREventModeSta]
  EVent/3(VTHC_FDCTHCLEventZSta_enum) -> [FDCTHCLEventZSta]
  [FDCTHCLEventZSta] -> Subsystem21/2(DataIn)
  Subsystem21/1(DataOut) -> VTHC_FDCTHCLEventZSta_enum/1
  EVent/4(VTHC_FDCTHCCLEVentZSta_enum) -> [FDCTHCCLEVentZSta]
  [FDCTHCCLEVentZSta] -> Subsystem22/2(DataIn)
  Subsystem22/1(DataOut) -> VTHC_FDCTHCCLEVentZSta_enum/1
  EVent/5(VTHC_FDCTHCREventZSta_enum) -> [FDCTHCREventZSta]
  [FDCTHCREventZSta] -> Subsystem23/2(DataIn)
  Subsystem23/1(DataOut) -> VTHC_FDCTHCREventZSta_enum/1
  Subsystem24/1(DataOut) -> VTHC_FDCTHCCREVentZSta_enum/1
  [FDCTHCCREVentZSta] -> Subsystem24/2(DataIn)
  EVent/6(VTHC_FDCTHCCREVentZSta_enum) -> [FDCTHCCREVentZSta]
  [FDCTHCLEventYSta] -> Subsystem25/2(DataIn)
  Subsystem25/1(DataOut) -> VTHC_FDCTHCLEventYSta_enum/1
  EVent/7(VTHC_FDCTHCLEventYSta_enum) -> [FDCTHCLEventYSta]
  EVent/8(VTHC_FDCTHCLVentEN_flg) -> [LVentEN]
  [LVentEN] -> Subsystem26/2(DataIn)
  Subsystem26/1(DataOut) -> Switch25/1
  EVent/9(VTHC_FDCTHCCLEVentYSta_enum) -> [FDCTHCCLEVentYSta]
  [FDCTHCCLEVentYSta] -> Subsystem27/2(DataIn)
  Subsystem27/1(DataOut) -> VTHC_FDCTHCCLEVentYSta_enum/1
  EVent/10(VTHC_FDCTHCCLVentEN_flg) -> [CLVentEN]
  Subsystem28/1(DataOut) -> Switch26/1
  [CLVentEN] -> Subsystem28/2(DataIn)
  EVent/11(VTHC_FDCTHCREventYSta_enum) -> [FDCTHCREventYSta]
  Subsystem29/1(DataOut) -> VTHC_FDCTHCREventYSta_enum/1
  [FDCTHCREventYSta] -> Subsystem29/2(DataIn)
  EVent/12(VTHC_FDCTHCRVentEN_flg) -> [RVentEN]
  Subsystem30/1(DataOut) -> Switch27/1
  [RVentEN] -> Subsystem30/2(DataIn)
  [FDCTHCCREVentYSta] -> Subsystem31/2(DataIn)
  Subsystem31/1(DataOut) -> VTHC_FDCTHCCREVentYSta_enum/1
  EVent/13(VTHC_FDCTHCCREVentYSta_enum) -> [FDCTHCCREVentYSta]
  EVent/14(VTHC_FDCTHCCRVentEN_flg) -> [CRVentEN]
  Subsystem32/1(DataOut) -> Switch28/1
  [CRVentEN] -> Subsystem32/2(DataIn)
  Logical Operator22/1 -> EVent/1(fInitial)
  [fInitial] -> Logical Operator22/2
  [Loading] -> Logical Operator27/1
  Logical Operator27/1 -> Logical Operator22/1
  Data Type Conversion1/1 -> Switch12/1
  Data Type Conversion6/1 -> Chart/71(EEP_ACModeMem)
  Data Type Conversion8/1 -> Chart/72(EEP_Face)
  Data Type Conversion9/1 -> Chart/73(EEP_Foot)
  Data Type Conversion44/1 -> Chart/74(EEP_Frost)
  Data Type Conversion45/1 -> Chart/75(EEP_FaceM)
  Data Type Conversion46/1 -> Chart/76(EEP_FootM)
  Data Type Conversion47/1 -> Chart/77(EEP_CCUSyncSts)
  Data Type Conversion48/1 -> Chart/78(EEP_sigRecircSt)
  Data Type Conversion49/1 -> Chart/79(EEP_RecAutoFlg)
  Data Type Conversion50/1 -> Chart/80(EEP_AirIntenZone1M)
  Data Type Conversion51/1 -> Chart/81(EEP_fdefog)
  Logical Operator9/1 -> Logical Operator21/1
  [VINP_CANMsgValidIVI2_flg] -> Switch21/2
  VINP_IVIFGSAirIntCmd_enum/1 -> Switch21/1
  Switch21/1 -> VALUE_TYPE_FDCFGSAirIntSta/6(SettingIn)
  Data Type Conversion7/1 -> Switch21/3
  Constant67/1 -> Data Type Conversion7/1
  [VINP_CANMsgValidIVI2_flg] -> EVent/30(VINP_CANMsgValidIVI2_flg)
  [ZLSetTP] -> Switch22/3
  [ZRSetTP] -> Switch22/1
  Constant68/1 -> Switch22/2
  Switch22/1 -> [Z1SetTP]
  VINP_HMIZLSetTPCmd_flg/1 -> HMISwitchReceive/1(VINP_HMIZLSetTPCmd_flg)
  VINP_HMIZLSetTMCmd_flg/1 -> HMISwitchReceive1/1(VINP_HMIZLSetTMCmd_flg)
  VINP_HMIZRSetTPCmd_flg/1 -> HMISwitchReceive2/1(VINP_HMIZRSetTPCmd_flg)
  VINP_HMIZRSetTMCmd_flg/1 -> HMISwitchReceive3/1(VINP_HMIZRSetTMCmd_flg)
  Switch30/1 -> [Z2SetTP]
  Constant69/1 -> Switch30/2
  [ZRSetTP] -> Switch30/3
  [ZLSetTP] -> Switch30/1
  [ZLSetTM] -> Switch32/1
  [ZRSetTM] -> Switch32/3
  Constant110/1 -> Switch32/2
  Switch32/1 -> [Z2SetTM]
  Switch31/1 -> [Z1SetTM]
  Constant70/1 -> Switch31/2
  [ZRSetTM] -> Switch31/1
  [ZLSetTM] -> Switch31/3
  Constant116/1 -> Chart/95(KTHC_WDZ11Face_flg)
  Constant114/1 -> Chart/96(KTHC_WDZ11Foot_flg)
  Constant115/1 -> Chart/97(KTHC_WDZ11Frost_flg)
  Constant119/1 -> Chart/98(KTHC_WDZ12Face_flg)
  Constant117/1 -> Chart/99(KTHC_WDZ12Foot_flg)
  Constant118/1 -> Chart/100(KTHC_WDZ12Frost_flg)
  Constant111/1 -> Chart/101(KTHC_AutoWDTamb1_C)
  Constant112/1 -> Chart/102(KTHC_AutoWDTamb2_C)
  Constant113/1 -> Chart/103(KTHC_AutoWDTamb3_C)
  VINP_IVIQuickRefreshSta_flg/1 -> Chart/104(VINP_IVIQuickRefreshSta_flg)
  Data Type Conversion/1 -> CCUSyncSts/1
